simulink model "model"  (R2014a)
(part 3 of 3)

  Ответвление_от_ВЛ_110кВ_Дубовый_Лес___Островы_CN_429035693_110000_CN_296016627_110000/LConn1 -- "T_429035693__ПС_\"Островы\""/LConn1 -- Ответвление_от_ВЛ_110кВ_Дубовый_Лес___Островы_CN_429035693_110000_CN_296016647_110000/LConn1 -- Ответвление_от_ВЛ_110кВ_Дубовый_Лес___Островы_CN_429035693_110000_CN_262743896_110000/LConn1 -- Ответвление_от_ВЛ_110кВ_Дубовый_Лес___Островы_CN_429035693_110000_CN_59099213_110000/LConn1 -- Ответвление_от_ВЛ_110кВ_Дубовый_Лес___Островы_CN_429035693_110000_CN_41194024_110000/LConn1 -- Ответвление_от_ВЛ_110кВ_Дубовый_Лес___Островы_CN_429035693_110000_CN_429148816_110000/LConn1
  Ответвление_от_ВЛ_110кВ_Дубовый_Лес___Островы_CN_429035693_110000_CN_296016627_110000/LConn2 -- "T_429035693__ПС_\"Островы\""/LConn2 -- Ответвление_от_ВЛ_110кВ_Дубовый_Лес___Островы_CN_429035693_110000_CN_296016647_110000/LConn2 -- Ответвление_от_ВЛ_110кВ_Дубовый_Лес___Островы_CN_429035693_110000_CN_262743896_110000/LConn2 -- Ответвление_от_ВЛ_110кВ_Дубовый_Лес___Островы_CN_429035693_110000_CN_59099213_110000/LConn2 -- Ответвление_от_ВЛ_110кВ_Дубовый_Лес___Островы_CN_429035693_110000_CN_41194024_110000/LConn2 -- Ответвление_от_ВЛ_110кВ_Дубовый_Лес___Островы_CN_429035693_110000_CN_429148816_110000/LConn2
  Ответвление_от_ВЛ_110кВ_Дубовый_Лес___Островы_CN_429035693_110000_CN_296016627_110000/LConn3 -- "T_429035693__ПС_\"Островы\""/LConn3 -- Ответвление_от_ВЛ_110кВ_Дубовый_Лес___Островы_CN_429035693_110000_CN_296016647_110000/LConn3 -- Ответвление_от_ВЛ_110кВ_Дубовый_Лес___Островы_CN_429035693_110000_CN_262743896_110000/LConn3 -- Ответвление_от_ВЛ_110кВ_Дубовый_Лес___Островы_CN_429035693_110000_CN_59099213_110000/LConn3 -- Ответвление_от_ВЛ_110кВ_Дубовый_Лес___Островы_CN_429035693_110000_CN_41194024_110000/LConn3 -- Ответвление_от_ВЛ_110кВ_Дубовый_Лес___Островы_CN_429035693_110000_CN_429148816_110000/LConn3 -- bus12/LConn1
  "T_296016627__ПС_\"Мачулищи\""/LConn1 -- Ответвление_от_ВЛ_110кВ_Дубовый_Лес___Островы_CN_429035693_110000_CN_296016627_110000/RConn1
  "T_296016627__ПС_\"Мачулищи\""/LConn2 -- Ответвление_от_ВЛ_110кВ_Дубовый_Лес___Островы_CN_429035693_110000_CN_296016627_110000/RConn2
  Ответвление_от_ВЛ_110кВ_Дубовый_Лес___Островы_CN_429035693_110000_CN_296016627_110000/RConn3 -- "T_296016627__ПС_\"Мачулищи\""/LConn3 -- bus13/LConn1
  "T_296016647__ПС_\"Кожзавод\""/LConn1 -- Ответвление_от_ВЛ_110кВ_Дубовый_Лес___Островы_CN_429035693_110000_CN_296016647_110000/RConn1
  "T_296016647__ПС_\"Кожзавод\""/LConn2 -- Ответвление_от_ВЛ_110кВ_Дубовый_Лес___Островы_CN_429035693_110000_CN_296016647_110000/RConn2
  Ответвление_от_ВЛ_110кВ_Дубовый_Лес___Островы_CN_429035693_110000_CN_296016647_110000/RConn3 -- "T_296016647__ПС_\"Кожзавод\""/LConn3 -- bus14/LConn1
  T_262743896__/LConn1 -- Ответвление_от_ВЛ_110кВ_Дубовый_Лес___Островы_CN_429035693_110000_CN_262743896_110000/RConn1
  T_262743896__/LConn2 -- Ответвление_от_ВЛ_110кВ_Дубовый_Лес___Островы_CN_429035693_110000_CN_262743896_110000/RConn2
  Ответвление_от_ВЛ_110кВ_Дубовый_Лес___Островы_CN_429035693_110000_CN_262743896_110000/RConn3 -- T_262743896__/LConn3 -- bus15/LConn1
  "T_59099213__ПС_\"Юго_Запад\""/LConn1 -- Ответвление_от_ВЛ_110кВ_Дубовый_Лес___Островы_CN_429035693_110000_CN_59099213_110000/RConn1
  "T_59099213__ПС_\"Юго_Запад\""/LConn2 -- Ответвление_от_ВЛ_110кВ_Дубовый_Лес___Островы_CN_429035693_110000_CN_59099213_110000/RConn2
  Ответвление_от_ВЛ_110кВ_Дубовый_Лес___Островы_CN_429035693_110000_CN_59099213_110000/RConn3 -- "T_59099213__ПС_\"Юго_Запад\""/LConn3 -- bus16/LConn1
  "T_41194024__ПС_\"Курасовщина\""/LConn1 -- Ответвление_от_ВЛ_110кВ_Дубовый_Лес___Островы_CN_429035693_110000_CN_41194024_110000/RConn1
  "T_41194024__ПС_\"Курасовщина\""/LConn2 -- Ответвление_от_ВЛ_110кВ_Дубовый_Лес___Островы_CN_429035693_110000_CN_41194024_110000/RConn2
  Ответвление_от_ВЛ_110кВ_Дубовый_Лес___Островы_CN_429035693_110000_CN_41194024_110000/RConn3 -- "T_41194024__ПС_\"Курасовщина\""/LConn3 -- bus17/LConn1
  "T_429148816__ПС_\"Кока_кола\""/LConn1 -- Ответвление_от_ВЛ_110кВ_Дубовый_Лес___Островы_CN_429035693_110000_CN_429148816_110000/RConn1
  "T_429148816__ПС_\"Кока_кола\""/LConn2 -- Ответвление_от_ВЛ_110кВ_Дубовый_Лес___Островы_CN_429035693_110000_CN_429148816_110000/RConn2
  Ответвление_от_ВЛ_110кВ_Дубовый_Лес___Островы_CN_429035693_110000_CN_429148816_110000/RConn3 -- "T_429148816__ПС_\"Кока_кола\""/LConn3 -- bus18/LConn1
  T_310063635__/LConn1 -- _CN_310063635_110000_CN_310178136_110000/LConn1
  T_310063635__/LConn2 -- _CN_310063635_110000_CN_310178136_110000/LConn2
  _CN_310063635_110000_CN_310178136_110000/LConn3 -- T_310063635__/LConn3 -- bus19/LConn1
  _CN_310063635_110000_CN_310178136_110000/RConn1 -- T_310178136__/LConn1 -- _CN_245414984_110000_CN_310178136_110000/LConn1
  _CN_310063635_110000_CN_310178136_110000/RConn2 -- T_310178136__/LConn2 -- _CN_245414984_110000_CN_310178136_110000/LConn2
  _CN_310063635_110000_CN_310178136_110000/RConn3 -- T_310178136__/LConn3 -- _CN_245414984_110000_CN_310178136_110000/LConn3 -- bus20/LConn1
  T_299173918__/LConn1 -- _CN_299173918_110000_CN_240568902_110000/LConn1
  T_299173918__/LConn2 -- _CN_299173918_110000_CN_240568902_110000/LConn2
  _CN_299173918_110000_CN_240568902_110000/LConn3 -- T_299173918__/LConn3 -- bus21/LConn1
  T_240568902__/LConn1 -- _CN_299173918_110000_CN_240568902_110000/RConn1
  T_240568902__/LConn2 -- _CN_299173918_110000_CN_240568902_110000/RConn2
  _CN_299173918_110000_CN_240568902_110000/RConn3 -- T_240568902__/LConn3 -- bus22/LConn1
  _CN_287228165_110000_CN_287231999_110000/LConn1 -- T_287228165__/LConn1 -- _CN_287228165_110000_CN_130795400_110000/LConn1
  _CN_287228165_110000_CN_287231999_110000/LConn2 -- T_287228165__/LConn2 -- _CN_287228165_110000_CN_130795400_110000/LConn2
  _CN_287228165_110000_CN_287231999_110000/LConn3 -- T_287228165__/LConn3 -- _CN_287228165_110000_CN_130795400_110000/LConn3 -- bus23/LConn1
  T_287231999__/LConn1 -- _CN_287228165_110000_CN_287231999_110000/RConn1
  T_287231999__/LConn2 -- _CN_287228165_110000_CN_287231999_110000/RConn2
  _CN_287228165_110000_CN_287231999_110000/RConn3 -- T_287231999__/LConn3 -- bus24/LConn1
  T_130795400__/LConn1 -- _CN_287228165_110000_CN_130795400_110000/RConn1
  T_130795400__/LConn2 -- _CN_287228165_110000_CN_130795400_110000/RConn2
  _CN_287228165_110000_CN_130795400_110000/RConn3 -- T_130795400__/LConn3 -- bus25/LConn1
  T_237040560__/LConn1 -- _CN_237040560_110000_CN_235777846_110000/RConn1
  T_237040560__/LConn2 -- _CN_237040560_110000_CN_235777846_110000/RConn2
  _CN_237040560_110000_CN_235777846_110000/RConn3 -- T_237040560__/LConn3 -- bus26/LConn1
  T_302900770__/LConn1 -- _CN_302900770_110000_CN_314058489_110000/LConn1
  T_302900770__/LConn2 -- _CN_302900770_110000_CN_314058489_110000/LConn2
  _CN_302900770_110000_CN_314058489_110000/LConn3 -- T_302900770__/LConn3 -- bus27/LConn1
  T_314058489__/LConn1 -- _CN_302900770_110000_CN_314058489_110000/RConn1
  T_314058489__/LConn2 -- _CN_302900770_110000_CN_314058489_110000/RConn2
  _CN_302900770_110000_CN_314058489_110000/RConn3 -- T_314058489__/LConn3 -- bus28/LConn1
  _CN_288873564_110000_CN_299211088_110000/LConn1 -- T_288873564__/LConn1 -- _CN_288873564_110000_CN_288873859_110000/RConn1
  _CN_288873564_110000_CN_299211088_110000/LConn2 -- T_288873564__/LConn2 -- _CN_288873564_110000_CN_288873859_110000/RConn2
  _CN_288873564_110000_CN_299211088_110000/LConn3 -- T_288873564__/LConn3 -- _CN_288873564_110000_CN_288873859_110000/RConn3 -- bus29/LConn1
  T_299211088__/LConn1 -- _CN_288873564_110000_CN_299211088_110000/RConn1
  T_299211088__/LConn2 -- _CN_288873564_110000_CN_299211088_110000/RConn2
  _CN_288873564_110000_CN_299211088_110000/RConn3 -- T_299211088__/LConn3 -- bus30/LConn1
  "T_224125485__ПС_\"Волма\""/LConn1 -- _CN_224125485_110000_CN_429056529_110000/LConn1
  "T_224125485__ПС_\"Волма\""/LConn2 -- _CN_224125485_110000_CN_429056529_110000/LConn2
  _CN_224125485_110000_CN_429056529_110000/LConn3 -- "T_224125485__ПС_\"Волма\""/LConn3 -- bus31/LConn1
  "T_429056529__ПС_\"Сосны\""/LConn1 -- _CN_224125485_110000_CN_429056529_110000/RConn1
  "T_429056529__ПС_\"Сосны\""/LConn2 -- _CN_224125485_110000_CN_429056529_110000/RConn2
  _CN_224125485_110000_CN_429056529_110000/RConn3 -- "T_429056529__ПС_\"Сосны\""/LConn3 -- bus32/LConn1
  T_429361631__/LConn1 -- _CN_429361631_110000_CN_24423222_110000/LConn1
  T_429361631__/LConn2 -- _CN_429361631_110000_CN_24423222_110000/LConn2
  _CN_429361631_110000_CN_24423222_110000/LConn3 -- T_429361631__/LConn3 -- bus33/LConn1
  _CN_429361631_110000_CN_24423222_110000/RConn1 -- G_24423222_ТЭЦ_3/RConn1 -- _CN_417002086_110000_CN_24423222_110000/LConn1 -- _CN_399298484_110000_CN_24423222_110000/LConn1
  _CN_429361631_110000_CN_24423222_110000/RConn2 -- G_24423222_ТЭЦ_3/RConn2 -- _CN_417002086_110000_CN_24423222_110000/LConn2 -- _CN_399298484_110000_CN_24423222_110000/LConn2
  _CN_429361631_110000_CN_24423222_110000/RConn3 -- G_24423222_ТЭЦ_3/RConn3 -- _CN_417002086_110000_CN_24423222_110000/LConn3 -- _CN_399298484_110000_CN_24423222_110000/LConn3 -- bus34/LConn1
  _CN_151029302_110000_CN_229441506_110000/LConn1 -- T_151029302__ПС_17_«Сторожёвская»/LConn1 -- _CN_151029302_110000_CN_40551785_110000/LConn1 -- _CN_151029302_110000_CN_154490102_110000/LConn1 -- _CN_151029302_110000_CN_429372327_110000/LConn1 -- _CN_151029302_110000_CN_60131045_110000/LConn1
  _CN_151029302_110000_CN_229441506_110000/LConn2 -- T_151029302__ПС_17_«Сторожёвская»/LConn2 -- _CN_151029302_110000_CN_40551785_110000/LConn2 -- _CN_151029302_110000_CN_154490102_110000/LConn2 -- _CN_151029302_110000_CN_429372327_110000/LConn2 -- _CN_151029302_110000_CN_60131045_110000/LConn2
  _CN_151029302_110000_CN_229441506_110000/LConn3 -- T_151029302__ПС_17_«Сторожёвская»/LConn3 -- _CN_151029302_110000_CN_40551785_110000/LConn3 -- _CN_151029302_110000_CN_154490102_110000/LConn3 -- _CN_151029302_110000_CN_429372327_110000/LConn3 -- _CN_151029302_110000_CN_60131045_110000/LConn3 -- bus35/LConn1
  _CN_151029302_110000_CN_229441506_110000/RConn1 -- T_229441506_330000_/RConn1 -- _CN_229441505_110000_CN_229441506_110000/LConn1 -- L_229441506/LConn1
  _CN_151029302_110000_CN_229441506_110000/RConn2 -- T_229441506_330000_/RConn2 -- _CN_229441505_110000_CN_229441506_110000/LConn2 -- L_229441506/LConn2
  _CN_151029302_110000_CN_229441506_110000/RConn3 -- T_229441506_330000_/RConn3 -- _CN_229441505_110000_CN_229441506_110000/LConn3 -- L_229441506/LConn3 -- bus36/LConn1
  "T_40551785__ПС_\"Уручье\""/LConn1 -- _CN_151029302_110000_CN_40551785_110000/RConn1
  "T_40551785__ПС_\"Уручье\""/LConn2 -- _CN_151029302_110000_CN_40551785_110000/RConn2
  _CN_151029302_110000_CN_40551785_110000/RConn3 -- "T_40551785__ПС_\"Уручье\""/LConn3 -- bus37/LConn1
  G_154490102_/RConn1 -- _CN_151029302_110000_CN_154490102_110000/RConn1
  G_154490102_/RConn2 -- _CN_151029302_110000_CN_154490102_110000/RConn2
  _CN_151029302_110000_CN_154490102_110000/RConn3 -- G_154490102_/RConn3 -- bus38/LConn1
  "T_429372327__ПС_\"Дражня\""/LConn1 -- _CN_151029302_110000_CN_429372327_110000/RConn1
  "T_429372327__ПС_\"Дражня\""/LConn2 -- _CN_151029302_110000_CN_429372327_110000/RConn2
  _CN_151029302_110000_CN_429372327_110000/RConn3 -- "T_429372327__ПС_\"Дражня\""/LConn3 -- bus39/LConn1
  "T_60131045__ПС_\"Озерище\""/LConn1 -- _CN_151029302_110000_CN_60131045_110000/RConn1
  "T_60131045__ПС_\"Озерище\""/LConn2 -- _CN_151029302_110000_CN_60131045_110000/RConn2
  _CN_151029302_110000_CN_60131045_110000/RConn3 -- "T_60131045__ПС_\"Озерище\""/LConn3 -- bus40/LConn1
  _CN_300409914_110000_CN_364529034_110000/LConn1 -- T_300409914__/LConn1 -- _CN_300409914_110000_CN_247791024_110000/LConn1
  _CN_300409914_110000_CN_364529034_110000/LConn2 -- T_300409914__/LConn2 -- _CN_300409914_110000_CN_247791024_110000/LConn2
  _CN_300409914_110000_CN_364529034_110000/LConn3 -- T_300409914__/LConn3 -- _CN_300409914_110000_CN_247791024_110000/LConn3 -- bus41/LConn1
  T_364529034__/LConn1 -- _CN_300409914_110000_CN_364529034_110000/RConn1
  T_364529034__/LConn2 -- _CN_300409914_110000_CN_364529034_110000/RConn2
  _CN_300409914_110000_CN_364529034_110000/RConn3 -- T_364529034__/LConn3 -- bus42/LConn1
  _CN_300409914_110000_CN_247791024_110000/RConn1 -- "T_247791024__ПС_330кВ_\"Слуцк\""/RConn1 -- _CN_300183354_110000_CN_247791024_110000/LConn1 -- _CN_394798987_110000_CN_247791024_110000/LConn1 -- L_247791024/LConn1 -- _CN_310325079_110000_CN_247791024_110000/LConn1
  _CN_300409914_110000_CN_247791024_110000/RConn2 -- "T_247791024__ПС_330кВ_\"Слуцк\""/RConn2 -- _CN_300183354_110000_CN_247791024_110000/LConn2 -- _CN_394798987_110000_CN_247791024_110000/LConn2 -- L_247791024/LConn2 -- _CN_310325079_110000_CN_247791024_110000/LConn2
  _CN_300409914_110000_CN_247791024_110000/RConn3 -- "T_247791024__ПС_330кВ_\"Слуцк\""/RConn3 -- _CN_300183354_110000_CN_247791024_110000/LConn3 -- _CN_394798987_110000_CN_247791024_110000/LConn3 -- L_247791024/LConn3 -- bus43/LConn1 -- _CN_310325079_110000_CN_247791024_110000/LConn3
  _CN_171987005_110000_CN_173944054_110000/LConn1 -- T_171987005_330000;110000;fixme_/RConn1 -- L_171987005/LConn1
  _CN_171987005_110000_CN_173944054_110000/LConn2 -- T_171987005_330000;110000;fixme_/RConn2 -- L_171987005/LConn2
  _CN_171987005_110000_CN_173944054_110000/LConn3 -- T_171987005_330000;110000;fixme_/RConn3 -- L_171987005/LConn3 -- bus44/LConn1
  _CN_171987005_110000_CN_173944054_110000/RConn1 -- T_173944054__/LConn1 -- _CN_173944047_110000_CN_173944054_110000/LConn1
  _CN_171987005_110000_CN_173944054_110000/RConn2 -- T_173944054__/LConn2 -- _CN_173944047_110000_CN_173944054_110000/LConn2
  _CN_171987005_110000_CN_173944054_110000/RConn3 -- T_173944054__/LConn3 -- _CN_173944047_110000_CN_173944054_110000/LConn3 -- bus45/LConn1
  T_429929483__/LConn1 -- _CN_429929483_110000_CN_301229003_110000/LConn1
  T_429929483__/LConn2 -- _CN_429929483_110000_CN_301229003_110000/LConn2
  _CN_429929483_110000_CN_301229003_110000/LConn3 -- T_429929483__/LConn3 -- bus46/LConn1
  T_301229003__/LConn1 -- _CN_429929483_110000_CN_301229003_110000/RConn1
  T_301229003__/LConn2 -- _CN_429929483_110000_CN_301229003_110000/RConn2
  _CN_429929483_110000_CN_301229003_110000/RConn3 -- T_301229003__/LConn3 -- bus47/LConn1
  T_299231301__/LConn1 -- _CN_299231301_110000_CN_299226289_110000/LConn1
  T_299231301__/LConn2 -- _CN_299231301_110000_CN_299226289_110000/LConn2
  _CN_299231301_110000_CN_299226289_110000/LConn3 -- T_299231301__/LConn3 -- bus48/LConn1
  _CN_299231301_110000_CN_299226289_110000/RConn1 -- T_299226289__/LConn1 -- _CN_299226289_110000_CN_223342356_110000/LConn1
  _CN_299231301_110000_CN_299226289_110000/RConn2 -- T_299226289__/LConn2 -- _CN_299226289_110000_CN_223342356_110000/LConn2
  _CN_299231301_110000_CN_299226289_110000/RConn3 -- T_299226289__/LConn3 -- _CN_299226289_110000_CN_223342356_110000/LConn3 -- bus49/LConn1
  _CN_245414984_110000_CN_310178136_110000/RConn1 -- "T_245414984__Подстанция_330_кВ_\"Молодечно\""/RConn1 -- L_245414984/LConn1
  _CN_245414984_110000_CN_310178136_110000/RConn2 -- "T_245414984__Подстанция_330_кВ_\"Молодечно\""/RConn2 -- L_245414984/LConn2
  _CN_245414984_110000_CN_310178136_110000/RConn3 -- "T_245414984__Подстанция_330_кВ_\"Молодечно\""/RConn3 -- L_245414984/LConn3 -- bus50/LConn1
  T_263648841__/LConn1 -- _CN_263648841_110000_CN_268654506_110000/LConn1
  T_263648841__/LConn2 -- _CN_263648841_110000_CN_268654506_110000/LConn2
  _CN_263648841_110000_CN_268654506_110000/LConn3 -- T_263648841__/LConn3 -- bus51/LConn1
  T_268654506__/LConn1 -- _CN_263648841_110000_CN_268654506_110000/RConn1
  T_268654506__/LConn2 -- _CN_263648841_110000_CN_268654506_110000/RConn2
  _CN_263648841_110000_CN_268654506_110000/RConn3 -- T_268654506__/LConn3 -- bus52/LConn1
  _CN_302733791_110000_CN_302726346_110000/LConn1 -- T_302733791__/LConn1 -- _CN_302733791_110000_CN_302734379_110000/LConn1
  _CN_302733791_110000_CN_302726346_110000/LConn2 -- T_302733791__/LConn2 -- _CN_302733791_110000_CN_302734379_110000/LConn2
  _CN_302733791_110000_CN_302726346_110000/LConn3 -- T_302733791__/LConn3 -- _CN_302733791_110000_CN_302734379_110000/LConn3 -- bus53/LConn1
  T_302726346_110000_Северная/LConn1 -- _CN_302733791_110000_CN_302726346_110000/RConn1
  T_302726346_110000_Северная/LConn2 -- _CN_302733791_110000_CN_302726346_110000/RConn2
  _CN_302733791_110000_CN_302726346_110000/RConn3 -- T_302726346_110000_Северная/LConn3 -- bus54/LConn1
  T_302734379__/LConn1 -- _CN_302733791_110000_CN_302734379_110000/RConn1
  T_302734379__/LConn2 -- _CN_302733791_110000_CN_302734379_110000/RConn2
  _CN_302733791_110000_CN_302734379_110000/RConn3 -- T_302734379__/LConn3 -- bus55/LConn1
  _CN_288267865_110000_CN_295775463_110000/LConn1 -- T_288267865__/LConn1 -- _CN_288267865_110000_CN_289493943_110000/LConn1 -- _CN_288267865_110000_CN_289501225_110000/LConn1
  _CN_288267865_110000_CN_295775463_110000/LConn2 -- T_288267865__/LConn2 -- _CN_288267865_110000_CN_289493943_110000/LConn2 -- _CN_288267865_110000_CN_289501225_110000/LConn2
  _CN_288267865_110000_CN_295775463_110000/LConn3 -- T_288267865__/LConn3 -- _CN_288267865_110000_CN_289493943_110000/LConn3 -- _CN_288267865_110000_CN_289501225_110000/LConn3 -- bus56/LConn1
  T_295775463__/LConn1 -- _CN_288267865_110000_CN_295775463_110000/RConn1
  T_295775463__/LConn2 -- _CN_288267865_110000_CN_295775463_110000/RConn2
  _CN_288267865_110000_CN_295775463_110000/RConn3 -- T_295775463__/LConn3 -- bus57/LConn1
  _CN_288267865_110000_CN_289493943_110000/RConn1 -- T_289493943__РЭС/LConn1 -- _CN_289501225_110000_CN_289493943_110000/LConn1
  _CN_288267865_110000_CN_289493943_110000/RConn2 -- T_289493943__РЭС/LConn2 -- _CN_289501225_110000_CN_289493943_110000/LConn2
  _CN_288267865_110000_CN_289493943_110000/RConn3 -- T_289493943__РЭС/LConn3 -- _CN_289501225_110000_CN_289493943_110000/LConn3 -- bus58/LConn1
  _CN_288267865_110000_CN_289501225_110000/RConn1 -- T_289501225__/LConn1 -- _CN_289501225_110000_CN_289493943_110000/RConn1
  _CN_288267865_110000_CN_289501225_110000/RConn2 -- T_289501225__/LConn2 -- _CN_289501225_110000_CN_289493943_110000/RConn2
  _CN_288267865_110000_CN_289501225_110000/RConn3 -- T_289501225__/LConn3 -- _CN_289501225_110000_CN_289493943_110000/RConn3 -- bus59/LConn1
  "T_255157340__Stacja_elektroenergetyczna_110kV_\"Hołowczyce\""/LConn1 -- 110_kV_Hołowczyce___Janów_Podlaski_CN_255157340_110000_CN_110512784_110000/LConn1
  "T_255157340__Stacja_elektroenergetyczna_110kV_\"Hołowczyce\""/LConn2 -- 110_kV_Hołowczyce___Janów_Podlaski_CN_255157340_110000_CN_110512784_110000/LConn2
  110_kV_Hołowczyce___Janów_Podlaski_CN_255157340_110000_CN_110512784_110000/LConn3 -- "T_255157340__Stacja_elektroenergetyczna_110kV_\"Hołowczyce\""/LConn3 -- bus60/LConn1
  110_kV_Hołowczyce___Janów_Podlaski_CN_255157340_110000_CN_110512784_110000/RConn1 -- "T_110512784__Stacja_elektroenergetyczna_110kV_\"Janów_Podlaski\""/LConn1 -- 110_kV_Wólka_Dobryńska___Janów_Podlaski_CN_110512784_110000_CN_108158175_110000/LConn1
  110_kV_Hołowczyce___Janów_Podlaski_CN_255157340_110000_CN_110512784_110000/RConn2 -- "T_110512784__Stacja_elektroenergetyczna_110kV_\"Janów_Podlaski\""/LConn2 -- 110_kV_Wólka_Dobryńska___Janów_Podlaski_CN_110512784_110000_CN_108158175_110000/LConn2
  110_kV_Hołowczyce___Janów_Podlaski_CN_255157340_110000_CN_110512784_110000/RConn3 -- "T_110512784__Stacja_elektroenergetyczna_110kV_\"Janów_Podlaski\""/LConn3 -- 110_kV_Wólka_Dobryńska___Janów_Podlaski_CN_110512784_110000_CN_108158175_110000/LConn3 -- bus61/LConn1
  _CN_310325079_110000_CN_300419261_110000/LConn1 -- T_310325079__ПС_110_кВ_«Копыль»/LConn1 -- _CN_310325079_110000_CN_247791024_110000/RConn1 -- _CN_310325079_110000_CN_300416246_110000/LConn1
  _CN_310325079_110000_CN_300419261_110000/LConn2 -- T_310325079__ПС_110_кВ_«Копыль»/LConn2 -- _CN_310325079_110000_CN_247791024_110000/RConn2 -- _CN_310325079_110000_CN_300416246_110000/LConn2
  _CN_310325079_110000_CN_300419261_110000/LConn3 -- T_310325079__ПС_110_кВ_«Копыль»/LConn3 -- _CN_310325079_110000_CN_247791024_110000/RConn3 -- _CN_310325079_110000_CN_300416246_110000/LConn3 -- bus62/LConn1
  "T_300419261__ПС_110_кВ_\"Терасполь\""/LConn1 -- _CN_310325079_110000_CN_300419261_110000/RConn1
  "T_300419261__ПС_110_кВ_\"Терасполь\""/LConn2 -- _CN_310325079_110000_CN_300419261_110000/RConn2
  _CN_310325079_110000_CN_300419261_110000/RConn3 -- "T_300419261__ПС_110_кВ_\"Терасполь\""/LConn3 -- bus63/LConn1
  _CN_310325079_110000_CN_300416246_110000/RConn1 -- T_300416246__/LConn1 -- _CN_300416246_110000_CN_275034427_110000/LConn1
  _CN_310325079_110000_CN_300416246_110000/RConn2 -- T_300416246__/LConn2 -- _CN_300416246_110000_CN_275034427_110000/LConn2
  _CN_310325079_110000_CN_300416246_110000/RConn3 -- T_300416246__/LConn3 -- _CN_300416246_110000_CN_275034427_110000/LConn3 -- bus64/LConn1
  T_299972194__/LConn1 -- _CN_299972194_110000_CN_299960721_110000/LConn1
  T_299972194__/LConn2 -- _CN_299972194_110000_CN_299960721_110000/LConn2
  _CN_299972194_110000_CN_299960721_110000/LConn3 -- T_299972194__/LConn3 -- bus65/LConn1
  T_299960721__/LConn1 -- _CN_299972194_110000_CN_299960721_110000/RConn1
  T_299960721__/LConn2 -- _CN_299972194_110000_CN_299960721_110000/RConn2
  _CN_299972194_110000_CN_299960721_110000/RConn3 -- T_299960721__/LConn3 -- bus66/LConn1
  _CN_417002086_110000_CN_429868839_110000/LConn1 -- "T_417002086_110000_ПС_\"Корзюки\""/LConn1 -- _CN_417002086_110000_CN_24423222_110000/RConn1 -- _CN_417002086_110000_CN_429740435_110000/LConn1 -- _CN_417002086_110000_CN_429148815_110000/LConn1
  _CN_417002086_110000_CN_429868839_110000/LConn2 -- "T_417002086_110000_ПС_\"Корзюки\""/LConn2 -- _CN_417002086_110000_CN_24423222_110000/RConn2 -- _CN_417002086_110000_CN_429740435_110000/LConn2 -- _CN_417002086_110000_CN_429148815_110000/LConn2
  _CN_417002086_110000_CN_429868839_110000/LConn3 -- "T_417002086_110000_ПС_\"Корзюки\""/LConn3 -- _CN_417002086_110000_CN_24423222_110000/RConn3 -- _CN_417002086_110000_CN_429740435_110000/LConn3 -- _CN_417002086_110000_CN_429148815_110000/LConn3 -- bus67/LConn1
  T_429868839__/LConn1 -- _CN_417002086_110000_CN_429868839_110000/RConn1
  T_429868839__/LConn2 -- _CN_417002086_110000_CN_429868839_110000/RConn2
  _CN_417002086_110000_CN_429868839_110000/RConn3 -- T_429868839__/LConn3 -- bus68/LConn1
  T_429740435__/LConn1 -- _CN_417002086_110000_CN_429740435_110000/RConn1
  T_429740435__/LConn2 -- _CN_417002086_110000_CN_429740435_110000/RConn2
  _CN_417002086_110000_CN_429740435_110000/RConn3 -- T_429740435__/LConn3 -- bus69/LConn1
  T_429148815__/LConn1 -- _CN_417002086_110000_CN_429148815_110000/RConn1
  T_429148815__/LConn2 -- _CN_417002086_110000_CN_429148815_110000/RConn2
  _CN_417002086_110000_CN_429148815_110000/RConn3 -- T_429148815__/LConn3 -- bus70/LConn1
  _CN_301876843_110000_CN_296183529_110000/LConn1 -- T_301876843__/LConn1 -- _CN_301876843_110000_CN_192882077_110000/LConn1
  _CN_301876843_110000_CN_296183529_110000/LConn2 -- T_301876843__/LConn2 -- _CN_301876843_110000_CN_192882077_110000/LConn2
  _CN_301876843_110000_CN_296183529_110000/LConn3 -- T_301876843__/LConn3 -- _CN_301876843_110000_CN_192882077_110000/LConn3 -- bus71/LConn1
  T_296183529__/LConn1 -- _CN_301876843_110000_CN_296183529_110000/RConn1
  T_296183529__/LConn2 -- _CN_301876843_110000_CN_296183529_110000/RConn2
  _CN_301876843_110000_CN_296183529_110000/RConn3 -- T_296183529__/LConn3 -- bus72/LConn1
  _CN_301876843_110000_CN_192882077_110000/RConn1 -- T_192882077__/RConn1 -- L_192882077/LConn1
  _CN_301876843_110000_CN_192882077_110000/RConn2 -- T_192882077__/RConn2 -- L_192882077/LConn2
  _CN_301876843_110000_CN_192882077_110000/RConn3 -- T_192882077__/RConn3 -- L_192882077/LConn3 -- bus73/LConn1
  _CN_222038644_110000_CN_429035699_110000/LConn1 -- "T_222038644__ПС_\"Свислочь\""/LConn1 -- _CN_222038644_110000_CN_226901999_110000/LConn1 -- _CN_222038644_110000_CN_299263429_110000/LConn1
  _CN_222038644_110000_CN_429035699_110000/LConn2 -- "T_222038644__ПС_\"Свислочь\""/LConn2 -- _CN_222038644_110000_CN_226901999_110000/LConn2 -- _CN_222038644_110000_CN_299263429_110000/LConn2
  _CN_222038644_110000_CN_429035699_110000/LConn3 -- "T_222038644__ПС_\"Свислочь\""/LConn3 -- _CN_222038644_110000_CN_226901999_110000/LConn3 -- _CN_222038644_110000_CN_299263429_110000/LConn3 -- bus74/LConn1
  _CN_222038644_110000_CN_429035699_110000/RConn1 -- "T_429035699__ПС_\"СУ_ТЭЦ_5\""/LConn1 -- _CN_299263429_110000_CN_429035699_110000/LConn1
  _CN_222038644_110000_CN_429035699_110000/RConn2 -- "T_429035699__ПС_\"СУ_ТЭЦ_5\""/LConn2 -- _CN_299263429_110000_CN_429035699_110000/LConn2
  _CN_222038644_110000_CN_429035699_110000/RConn3 -- "T_429035699__ПС_\"СУ_ТЭЦ_5\""/LConn3 -- _CN_299263429_110000_CN_429035699_110000/LConn3 -- bus75/LConn1
  "T_226901999__ПС_\"Руденск\""/LConn1 -- _CN_222038644_110000_CN_226901999_110000/RConn1
  "T_226901999__ПС_\"Руденск\""/LConn2 -- _CN_222038644_110000_CN_226901999_110000/RConn2
  _CN_222038644_110000_CN_226901999_110000/RConn3 -- "T_226901999__ПС_\"Руденск\""/LConn3 -- bus76/LConn1
  _CN_222038644_110000_CN_299263429_110000/RConn1 -- T_299263429__/LConn1 -- _CN_299263429_110000_CN_429035699_110000/RConn1
  _CN_222038644_110000_CN_299263429_110000/RConn2 -- T_299263429__/LConn2 -- _CN_299263429_110000_CN_429035699_110000/RConn2
  _CN_222038644_110000_CN_299263429_110000/RConn3 -- T_299263429__/LConn3 -- _CN_299263429_110000_CN_429035699_110000/RConn3 -- bus77/LConn1
  T_296414541__/LConn1 -- _CN_296414541_110000_CN_289722224_110000/LConn1
  T_296414541__/LConn2 -- _CN_296414541_110000_CN_289722224_110000/LConn2
  _CN_296414541_110000_CN_289722224_110000/LConn3 -- T_296414541__/LConn3 -- bus78/LConn1
  _CN_296414541_110000_CN_289722224_110000/RConn1 -- T_289722224__/LConn1 -- _CN_289722224_110000_CN_25141415_110000/LConn1
  _CN_296414541_110000_CN_289722224_110000/RConn2 -- T_289722224__/LConn2 -- _CN_289722224_110000_CN_25141415_110000/LConn2
  _CN_296414541_110000_CN_289722224_110000/RConn3 -- T_289722224__/LConn3 -- _CN_289722224_110000_CN_25141415_110000/LConn3 -- bus79/LConn1
  T_294809961__/LConn1 -- _CN_294809961_110000_CN_287057886_110000/LConn1
  T_294809961__/LConn2 -- _CN_294809961_110000_CN_287057886_110000/LConn2
  _CN_294809961_110000_CN_287057886_110000/LConn3 -- T_294809961__/LConn3 -- bus80/LConn1
  T_287057886__/LConn1 -- _CN_294809961_110000_CN_287057886_110000/RConn1
  T_287057886__/LConn2 -- _CN_294809961_110000_CN_287057886_110000/RConn2
  _CN_294809961_110000_CN_287057886_110000/RConn3 -- T_287057886__/LConn3 -- bus81/LConn1
  T_34327162__/LConn1 -- _CN_34327162_110000_CN_177731028_110000/LConn1
  T_34327162__/LConn2 -- _CN_34327162_110000_CN_177731028_110000/LConn2
  _CN_34327162_110000_CN_177731028_110000/LConn3 -- T_34327162__/LConn3 -- bus82/LConn1
  _CN_34327162_110000_CN_177731028_110000/RConn1 -- T_177731028__/LConn1 -- ВЛ_110_кВ_Пилюки_Лозы_CN_89723141_110000_CN_177731028_110000/RConn1
  _CN_34327162_110000_CN_177731028_110000/RConn2 -- T_177731028__/LConn2 -- ВЛ_110_кВ_Пилюки_Лозы_CN_89723141_110000_CN_177731028_110000/RConn2
  _CN_34327162_110000_CN_177731028_110000/RConn3 -- T_177731028__/LConn3 -- ВЛ_110_кВ_Пилюки_Лозы_CN_89723141_110000_CN_177731028_110000/RConn3 -- bus83/LConn1
  T_194912891__Stacja_elektroenergetyczna_110_15_kV_Lubień/LConn1 -- Linia_110_kV_Włodawa___Lubień_CN_194912891_110000_CN_105490801_110000/LConn1
  T_194912891__Stacja_elektroenergetyczna_110_15_kV_Lubień/LConn2 -- Linia_110_kV_Włodawa___Lubień_CN_194912891_110000_CN_105490801_110000/LConn2
  Linia_110_kV_Włodawa___Lubień_CN_194912891_110000_CN_105490801_110000/LConn3 -- T_194912891__Stacja_elektroenergetyczna_110_15_kV_Lubień/LConn3 -- bus84/LConn1
  Linia_110_kV_Włodawa___Lubień_CN_194912891_110000_CN_105490801_110000/RConn1 -- T_105490801__Stacja_elektroenergetyczna_110_15_kV_Włodawa/LConn1 -- Linia_110_kV_Macoszyn___Włodawa_CN_194911376_110000_CN_105490801_110000/LConn1
  Linia_110_kV_Włodawa___Lubień_CN_194912891_110000_CN_105490801_110000/RConn2 -- T_105490801__Stacja_elektroenergetyczna_110_15_kV_Włodawa/LConn2 -- Linia_110_kV_Macoszyn___Włodawa_CN_194911376_110000_CN_105490801_110000/LConn2
  Linia_110_kV_Włodawa___Lubień_CN_194912891_110000_CN_105490801_110000/RConn3 -- T_105490801__Stacja_elektroenergetyczna_110_15_kV_Włodawa/LConn3 -- Linia_110_kV_Macoszyn___Włodawa_CN_194911376_110000_CN_105490801_110000/LConn3 -- bus85/LConn1
  T_230273156__/LConn1 -- _CN_230273156_110000_CN_230273164_110000/LConn1
  T_230273156__/LConn2 -- _CN_230273156_110000_CN_230273164_110000/LConn2
  _CN_230273156_110000_CN_230273164_110000/LConn3 -- T_230273156__/LConn3 -- bus86/LConn1
  T_230273164_110000_Подстанция_110_кВ_Южная/LConn1 -- _CN_230273156_110000_CN_230273164_110000/RConn1
  T_230273164_110000_Подстанция_110_кВ_Южная/LConn2 -- _CN_230273156_110000_CN_230273164_110000/RConn2
  _CN_230273156_110000_CN_230273164_110000/RConn3 -- T_230273164_110000_Подстанция_110_кВ_Южная/LConn3 -- bus87/LConn1
  "T_142803081__ПС_\"Заславль\""/LConn1 -- _CN_142803081_110000_CN_429035686_110000/LConn1
  "T_142803081__ПС_\"Заславль\""/LConn2 -- _CN_142803081_110000_CN_429035686_110000/LConn2
  _CN_142803081_110000_CN_429035686_110000/LConn3 -- "T_142803081__ПС_\"Заславль\""/LConn3 -- bus88/LConn1
  "T_429035686__ПС_\"Мехкарьер\""/LConn1 -- _CN_142803081_110000_CN_429035686_110000/RConn1
  "T_429035686__ПС_\"Мехкарьер\""/LConn2 -- _CN_142803081_110000_CN_429035686_110000/RConn2
  _CN_142803081_110000_CN_429035686_110000/RConn3 -- "T_429035686__ПС_\"Мехкарьер\""/LConn3 -- bus89/LConn1
  "T_108158175__Stacja_elektroenergetyczna_110kV_\"Wólka_Dobryńska\""/LConn1 -- 110_kV_Wólka_Dobryńska___Janów_Podlaski_CN_110512784_110000_CN_108158175_110000/RConn1
  "T_108158175__Stacja_elektroenergetyczna_110kV_\"Wólka_Dobryńska\""/LConn2 -- 110_kV_Wólka_Dobryńska___Janów_Podlaski_CN_110512784_110000_CN_108158175_110000/RConn2
  110_kV_Wólka_Dobryńska___Janów_Podlaski_CN_110512784_110000_CN_108158175_110000/RConn3 -- "T_108158175__Stacja_elektroenergetyczna_110kV_\"Wólka_Dobryńska\""/LConn3 -- bus90/LConn1
  "T_248455324__ПС_\"Атлант\""/LConn1 -- _CN_248455324_110000_CN_248452429_110000/LConn1
  "T_248455324__ПС_\"Атлант\""/LConn2 -- _CN_248455324_110000_CN_248452429_110000/LConn2
  _CN_248455324_110000_CN_248452429_110000/LConn3 -- "T_248455324__ПС_\"Атлант\""/LConn3 -- bus91/LConn1
  "T_248452429__ПС_\"Шабаны_2\""/LConn1 -- _CN_248455324_110000_CN_248452429_110000/RConn1
  "T_248452429__ПС_\"Шабаны_2\""/LConn2 -- _CN_248455324_110000_CN_248452429_110000/RConn2
  _CN_248455324_110000_CN_248452429_110000/RConn3 -- "T_248452429__ПС_\"Шабаны_2\""/LConn3 -- bus92/LConn1
  T_227158696__/LConn1 -- _CN_227158696_110000_CN_240810375_110000/LConn1
  T_227158696__/LConn2 -- _CN_227158696_110000_CN_240810375_110000/LConn2
  _CN_227158696_110000_CN_240810375_110000/LConn3 -- T_227158696__/LConn3 -- bus93/LConn1
  T_240810375__/LConn1 -- _CN_227158696_110000_CN_240810375_110000/RConn1
  T_240810375__/LConn2 -- _CN_227158696_110000_CN_240810375_110000/RConn2
  _CN_227158696_110000_CN_240810375_110000/RConn3 -- T_240810375__/LConn3 -- bus94/LConn1
  ВЛ_110_кВ_Лучники___Новое_Гутково_CN_373095383_110000_CN_300430643_110000/LConn1 -- T_373095383__/LConn1 -- ВЛ_110_кВ_Старые_Дороги___Новое_Гутково_CN_373095383_110000_CN_260356877_110000/LConn1
  ВЛ_110_кВ_Лучники___Новое_Гутково_CN_373095383_110000_CN_300430643_110000/LConn2 -- T_373095383__/LConn2 -- ВЛ_110_кВ_Старые_Дороги___Новое_Гутково_CN_373095383_110000_CN_260356877_110000/LConn2
  ВЛ_110_кВ_Лучники___Новое_Гутково_CN_373095383_110000_CN_300430643_110000/LConn3 -- T_373095383__/LConn3 -- ВЛ_110_кВ_Старые_Дороги___Новое_Гутково_CN_373095383_110000_CN_260356877_110000/LConn3 -- bus95/LConn1
  "T_300430643__ПС_110_кВ_\"Лучники\""/LConn1 -- ВЛ_110_кВ_Лучники___Новое_Гутково_CN_373095383_110000_CN_300430643_110000/RConn1
  "T_300430643__ПС_110_кВ_\"Лучники\""/LConn2 -- ВЛ_110_кВ_Лучники___Новое_Гутково_CN_373095383_110000_CN_300430643_110000/RConn2
  ВЛ_110_кВ_Лучники___Новое_Гутково_CN_373095383_110000_CN_300430643_110000/RConn3 -- "T_300430643__ПС_110_кВ_\"Лучники\""/LConn3 -- bus96/LConn1
  ВЛ_110_кВ_Старые_Дороги___Новое_Гутково_CN_373095383_110000_CN_260356877_110000/RConn1 -- T_260356877_750000;330000_Белорусская/RConn1 -- L_260356877/LConn1
  ВЛ_110_кВ_Старые_Дороги___Новое_Гутково_CN_373095383_110000_CN_260356877_110000/RConn2 -- T_260356877_750000;330000_Белорусская/RConn2 -- L_260356877/LConn2
  ВЛ_110_кВ_Старые_Дороги___Новое_Гутково_CN_373095383_110000_CN_260356877_110000/RConn3 -- T_260356877_750000;330000_Белорусская/RConn3 -- L_260356877/LConn3 -- bus97/LConn1
  T_223342356__/LConn1 -- _CN_299226289_110000_CN_223342356_110000/RConn1
  T_223342356__/LConn2 -- _CN_299226289_110000_CN_223342356_110000/RConn2
  _CN_299226289_110000_CN_223342356_110000/RConn3 -- T_223342356__/LConn3 -- bus98/LConn1
  T_409058996__/LConn1 -- ВЛ_Калийная___Уречье_110кВ_CN_409058996_110000_CN_232431375_110000/LConn1
  T_409058996__/LConn2 -- ВЛ_Калийная___Уречье_110кВ_CN_409058996_110000_CN_232431375_110000/LConn2
  ВЛ_Калийная___Уречье_110кВ_CN_409058996_110000_CN_232431375_110000/LConn3 -- T_409058996__/LConn3 -- bus99/LConn1
  T_232431375__/LConn1 -- ВЛ_Калийная___Уречье_110кВ_CN_409058996_110000_CN_232431375_110000/RConn1
  T_232431375__/LConn2 -- ВЛ_Калийная___Уречье_110кВ_CN_409058996_110000_CN_232431375_110000/RConn2
  ВЛ_Калийная___Уречье_110кВ_CN_409058996_110000_CN_232431375_110000/RConn3 -- T_232431375__/LConn3 -- bus100/LConn1
  _CN_283245238_110000_CN_235391296_110000/LConn1 -- T_283245238_330000_/RConn1 -- L_283245238/LConn1
  _CN_283245238_110000_CN_235391296_110000/LConn2 -- T_283245238_330000_/RConn2 -- L_283245238/LConn2
  _CN_283245238_110000_CN_235391296_110000/LConn3 -- T_283245238_330000_/RConn3 -- L_283245238/LConn3 -- bus101/LConn1
  _CN_283245238_110000_CN_235391296_110000/RConn1 -- T_235391296__/LConn1 -- _CN_235777846_110000_CN_235391296_110000/RConn1
  _CN_283245238_110000_CN_235391296_110000/RConn2 -- T_235391296__/LConn2 -- _CN_235777846_110000_CN_235391296_110000/RConn2
  _CN_283245238_110000_CN_235391296_110000/RConn3 -- T_235391296__/LConn3 -- _CN_235777846_110000_CN_235391296_110000/RConn3 -- bus102/LConn1
  "T_275034427__ПС_\"Красная_Слобода\""/LConn1 -- _CN_300416246_110000_CN_275034427_110000/RConn1
  "T_275034427__ПС_\"Красная_Слобода\""/LConn2 -- _CN_300416246_110000_CN_275034427_110000/RConn2
  _CN_300416246_110000_CN_275034427_110000/RConn3 -- "T_275034427__ПС_\"Красная_Слобода\""/LConn3 -- bus103/LConn1
  T_309889740__/LConn1 -- _CN_309889740_110000_CN_25141415_110000/LConn1
  T_309889740__/LConn2 -- _CN_309889740_110000_CN_25141415_110000/LConn2
  _CN_309889740_110000_CN_25141415_110000/LConn3 -- T_309889740__/LConn3 -- bus104/LConn1
  _CN_309889740_110000_CN_25141415_110000/RConn1 -- G_25141415_Берёзовская_ГРЭС/RConn1 -- _CN_289722224_110000_CN_25141415_110000/RConn1 -- 220kV_Białystok___Рось_CN_216254873_220000_CN_25141415_110000/LConn1
  _CN_309889740_110000_CN_25141415_110000/RConn2 -- G_25141415_Берёзовская_ГРЭС/RConn2 -- _CN_289722224_110000_CN_25141415_110000/RConn2 -- 220kV_Białystok___Рось_CN_216254873_220000_CN_25141415_110000/LConn2
  _CN_309889740_110000_CN_25141415_110000/RConn3 -- G_25141415_Берёзовская_ГРЭС/RConn3 -- _CN_289722224_110000_CN_25141415_110000/RConn3 -- 220kV_Białystok___Рось_CN_216254873_220000_CN_25141415_110000/LConn3 -- bus105/LConn1
  _CN_230054607_110000_CN_271931809_110000/LConn1 -- T_230054607__Барановичи_330/RConn4 -- _CN_230054607_110000_CN_296408783_110000/LConn1 -- _CN_230054607_110000_CN_230054608_110000/LConn1 -- L_230054607/LConn1
  _CN_230054607_110000_CN_271931809_110000/LConn2 -- T_230054607__Барановичи_330/RConn5 -- _CN_230054607_110000_CN_296408783_110000/LConn2 -- _CN_230054607_110000_CN_230054608_110000/LConn2 -- L_230054607/LConn2
  _CN_230054607_110000_CN_271931809_110000/LConn3 -- T_230054607__Барановичи_330/RConn6 -- _CN_230054607_110000_CN_296408783_110000/LConn3 -- _CN_230054607_110000_CN_230054608_110000/LConn3 -- L_230054607/LConn3 -- bus106/LConn1
  T_271931809__/LConn1 -- _CN_230054607_110000_CN_271931809_110000/RConn1
  T_271931809__/LConn2 -- _CN_230054607_110000_CN_271931809_110000/RConn2
  _CN_230054607_110000_CN_271931809_110000/RConn3 -- T_271931809__/LConn3 -- bus107/LConn1
  T_296408783__/LConn1 -- _CN_230054607_110000_CN_296408783_110000/RConn1
  T_296408783__/LConn2 -- _CN_230054607_110000_CN_296408783_110000/RConn2
  _CN_230054607_110000_CN_296408783_110000/RConn3 -- T_296408783__/LConn3 -- bus108/LConn1
  _CN_230054607_110000_CN_230054608_110000/RConn1 -- T_230054608__Барановичи_220/RConn1 -- _CN_230054608_110000_CN_230054609_110000/LConn1 -- L_230054608/LConn1
  _CN_230054607_110000_CN_230054608_110000/RConn2 -- T_230054608__Барановичи_220/RConn2 -- _CN_230054608_110000_CN_230054609_110000/LConn2 -- L_230054608/LConn2
  _CN_230054607_110000_CN_230054608_110000/RConn3 -- T_230054608__Барановичи_220/RConn3 -- _CN_230054608_110000_CN_230054609_110000/LConn3 -- L_230054608/LConn3 -- bus109/LConn1
  T_230054609__/LConn1 -- _CN_230054608_110000_CN_230054609_110000/RConn1
  T_230054609__/LConn2 -- _CN_230054608_110000_CN_230054609_110000/RConn2
  _CN_230054608_110000_CN_230054609_110000/RConn3 -- T_230054609__/LConn3 -- bus110/LConn1
  T_298978939__/LConn1 -- _CN_298978939_110000_CN_280269221_110000/LConn1
  T_298978939__/LConn2 -- _CN_298978939_110000_CN_280269221_110000/LConn2
  _CN_298978939_110000_CN_280269221_110000/LConn3 -- T_298978939__/LConn3 -- bus111/LConn1
  T_280269221__/LConn1 -- _CN_298978939_110000_CN_280269221_110000/RConn1
  T_280269221__/LConn2 -- _CN_298978939_110000_CN_280269221_110000/RConn2
  _CN_298978939_110000_CN_280269221_110000/RConn3 -- T_280269221__/LConn3 -- bus112/LConn1
  _CN_173944047_110000_CN_311242021_110000/LConn1 -- T_173944047__/LConn1 -- _CN_173944047_110000_CN_173944054_110000/RConn1
  _CN_173944047_110000_CN_311242021_110000/LConn2 -- T_173944047__/LConn2 -- _CN_173944047_110000_CN_173944054_110000/RConn2
  _CN_173944047_110000_CN_311242021_110000/LConn3 -- T_173944047__/LConn3 -- _CN_173944047_110000_CN_173944054_110000/RConn3 -- bus113/LConn1
  T_311242021__/LConn1 -- _CN_173944047_110000_CN_311242021_110000/RConn1
  T_311242021__/LConn2 -- _CN_173944047_110000_CN_311242021_110000/RConn2
  _CN_173944047_110000_CN_311242021_110000/RConn3 -- T_311242021__/LConn3 -- bus114/LConn1
  T_192951026__/LConn1 -- _CN_192951026_110000_CN_201828730_110000/LConn1
  T_192951026__/LConn2 -- _CN_192951026_110000_CN_201828730_110000/LConn2
  _CN_192951026_110000_CN_201828730_110000/LConn3 -- T_192951026__/LConn3 -- bus115/LConn1
  _CN_192951026_110000_CN_201828730_110000/RConn1 -- T_201828730_330000_/RConn4 -- _CN_325933845_110000_CN_201828730_110000/LConn1 -- L_201828730/LConn1
  _CN_192951026_110000_CN_201828730_110000/RConn2 -- T_201828730_330000_/RConn5 -- _CN_325933845_110000_CN_201828730_110000/LConn2 -- L_201828730/LConn2
  _CN_192951026_110000_CN_201828730_110000/RConn3 -- T_201828730_330000_/RConn6 -- _CN_325933845_110000_CN_201828730_110000/LConn3 -- L_201828730/LConn3 -- bus116/LConn1
  T_168120565__/LConn1 -- _CN_168120565_110000_CN_199487387_110000/LConn1
  T_168120565__/LConn2 -- _CN_168120565_110000_CN_199487387_110000/LConn2
  _CN_168120565_110000_CN_199487387_110000/LConn3 -- T_168120565__/LConn3 -- bus117/LConn1
  T_199487387__/LConn1 -- _CN_168120565_110000_CN_199487387_110000/RConn1
  T_199487387__/LConn2 -- _CN_168120565_110000_CN_199487387_110000/RConn2
  _CN_168120565_110000_CN_199487387_110000/RConn3 -- T_199487387__/LConn3 -- bus118/LConn1
  T_223761142__ПС_110_кВ_Гродненская_ГЭС/LConn1 -- _CN_223761142_110000_CN_177731027_110000/LConn1
  T_223761142__ПС_110_кВ_Гродненская_ГЭС/LConn2 -- _CN_223761142_110000_CN_177731027_110000/LConn2
  _CN_223761142_110000_CN_177731027_110000/LConn3 -- T_223761142__ПС_110_кВ_Гродненская_ГЭС/LConn3 -- bus119/LConn1
  T_177731027__/LConn1 -- _CN_223761142_110000_CN_177731027_110000/RConn1
  T_177731027__/LConn2 -- _CN_223761142_110000_CN_177731027_110000/RConn2
  _CN_223761142_110000_CN_177731027_110000/RConn3 -- T_177731027__/LConn3 -- bus120/LConn1
  "T_52763915__ПС_\"Лошица\""/LConn1 -- _CN_52763915_110000_CN_143993676_110000/LConn1
  "T_52763915__ПС_\"Лошица\""/LConn2 -- _CN_52763915_110000_CN_143993676_110000/LConn2
  _CN_52763915_110000_CN_143993676_110000/LConn3 -- "T_52763915__ПС_\"Лошица\""/LConn3 -- bus121/LConn1
  T_143993676__ПС_Минский_камвольный_комбинат/LConn1 -- _CN_52763915_110000_CN_143993676_110000/RConn1
  T_143993676__ПС_Минский_камвольный_комбинат/LConn2 -- _CN_52763915_110000_CN_143993676_110000/RConn2
  _CN_52763915_110000_CN_143993676_110000/RConn3 -- T_143993676__ПС_Минский_камвольный_комбинат/LConn3 -- bus122/LConn1
  _CN_325933845_110000_CN_201828730_110000/RConn1 -- T_325933845__/LConn1 -- _CN_325933845_110000_CN_166169945_110000/LConn1
  _CN_325933845_110000_CN_201828730_110000/RConn2 -- T_325933845__/LConn2 -- _CN_325933845_110000_CN_166169945_110000/LConn2
  _CN_325933845_110000_CN_201828730_110000/RConn3 -- T_325933845__/LConn3 -- _CN_325933845_110000_CN_166169945_110000/LConn3 -- bus123/LConn1
  _CN_325933845_110000_CN_166169945_110000/RConn1 -- T_166169945__/LConn1 -- _CN_166169945_110000_CN_88831410_110000/LConn1
  _CN_325933845_110000_CN_166169945_110000/RConn2 -- T_166169945__/LConn2 -- _CN_166169945_110000_CN_88831410_110000/LConn2
  _CN_325933845_110000_CN_166169945_110000/RConn3 -- T_166169945__/LConn3 -- _CN_166169945_110000_CN_88831410_110000/LConn3 -- bus124/LConn1
  _CN_230059286_110000_CN_230059305_110000/LConn1 -- T_230059286__/RConn1 -- L_230059286/LConn1
  _CN_230059286_110000_CN_230059305_110000/LConn2 -- T_230059286__/RConn2 -- L_230059286/LConn2
  _CN_230059286_110000_CN_230059305_110000/LConn3 -- T_230059286__/RConn3 -- L_230059286/LConn3 -- bus125/LConn1
  _CN_230059286_110000_CN_230059305_110000/RConn1 -- T_230059305_110000_Осташковичи/LConn1 -- _CN_230059305_110000_CN_282201051_110000/LConn1
  _CN_230059286_110000_CN_230059305_110000/RConn2 -- T_230059305_110000_Осташковичи/LConn2 -- _CN_230059305_110000_CN_282201051_110000/LConn2
  _CN_230059286_110000_CN_230059305_110000/RConn3 -- T_230059305_110000_Осташковичи/LConn3 -- _CN_230059305_110000_CN_282201051_110000/LConn3 -- bus126/LConn1
  T_366740253__/LConn1 -- _CN_366740253_110000_CN_262762815_110000/LConn1
  T_366740253__/LConn2 -- _CN_366740253_110000_CN_262762815_110000/LConn2
  _CN_366740253_110000_CN_262762815_110000/LConn3 -- T_366740253__/LConn3 -- bus127/LConn1
  T_262762815__/LConn1 -- _CN_366740253_110000_CN_262762815_110000/RConn1
  T_262762815__/LConn2 -- _CN_366740253_110000_CN_262762815_110000/RConn2
  _CN_366740253_110000_CN_262762815_110000/RConn3 -- T_262762815__/LConn3 -- bus128/LConn1
  T_282201051__Якимова_Слобода/LConn1 -- _CN_230059305_110000_CN_282201051_110000/RConn1
  T_282201051__Якимова_Слобода/LConn2 -- _CN_230059305_110000_CN_282201051_110000/RConn2
  _CN_230059305_110000_CN_282201051_110000/RConn3 -- T_282201051__Якимова_Слобода/LConn3 -- bus129/LConn1
  T_282200754_110000_Забродье/LConn1 -- _CN_282200754_110000_CN_286434280_110000/LConn1
  T_282200754_110000_Забродье/LConn2 -- _CN_282200754_110000_CN_286434280_110000/LConn2
  _CN_282200754_110000_CN_286434280_110000/LConn3 -- T_282200754_110000_Забродье/LConn3 -- bus130/LConn1
  T_286434280__/LConn1 -- _CN_282200754_110000_CN_286434280_110000/RConn1
  T_286434280__/LConn2 -- _CN_282200754_110000_CN_286434280_110000/RConn2
  _CN_282200754_110000_CN_286434280_110000/RConn3 -- T_286434280__/LConn3 -- bus131/LConn1
  _CN_300183354_110000_CN_247791024_110000/RConn1 -- T_300183354__/LConn1 -- _CN_300183354_110000_CN_300236667_110000/LConn1
  _CN_300183354_110000_CN_247791024_110000/RConn2 -- T_300183354__/LConn2 -- _CN_300183354_110000_CN_300236667_110000/LConn2
  _CN_300183354_110000_CN_247791024_110000/RConn3 -- T_300183354__/LConn3 -- _CN_300183354_110000_CN_300236667_110000/LConn3 -- bus132/LConn1
  T_300236667__/LConn1 -- _CN_300183354_110000_CN_300236667_110000/RConn1
  T_300236667__/LConn2 -- _CN_300183354_110000_CN_300236667_110000/RConn2
  _CN_300183354_110000_CN_300236667_110000/RConn3 -- T_300236667__/LConn3 -- bus133/LConn1
  T_108689220__/LConn1 -- _CN_108689220_110000_CN_295351112_110000/LConn1
  T_108689220__/LConn2 -- _CN_108689220_110000_CN_295351112_110000/LConn2
  _CN_108689220_110000_CN_295351112_110000/LConn3 -- T_108689220__/LConn3 -- bus134/LConn1
  _CN_108689220_110000_CN_295351112_110000/RConn1 -- T_295351112_330000_/LConn1 -- _CN_295351112_110000_CN_168037760_110000/LConn1
  _CN_108689220_110000_CN_295351112_110000/RConn2 -- T_295351112_330000_/LConn2 -- _CN_295351112_110000_CN_168037760_110000/LConn2
  _CN_108689220_110000_CN_295351112_110000/RConn3 -- T_295351112_330000_/LConn3 -- _CN_295351112_110000_CN_168037760_110000/LConn3 -- bus135/LConn1
  T_168037760__/LConn1 -- _CN_295351112_110000_CN_168037760_110000/RConn1
  T_168037760__/LConn2 -- _CN_295351112_110000_CN_168037760_110000/RConn2
  _CN_295351112_110000_CN_168037760_110000/RConn3 -- T_168037760__/LConn3 -- bus136/LConn1
  _CN_293851177_110000_CN_276283812_110000/LConn1 -- T_293851177__/LConn1 -- _CN_293851177_110000_CN_293845492_110000/LConn1
  _CN_293851177_110000_CN_276283812_110000/LConn2 -- T_293851177__/LConn2 -- _CN_293851177_110000_CN_293845492_110000/LConn2
  _CN_293851177_110000_CN_276283812_110000/LConn3 -- T_293851177__/LConn3 -- _CN_293851177_110000_CN_293845492_110000/LConn3 -- bus137/LConn1
  T_276283812__/LConn1 -- _CN_293851177_110000_CN_276283812_110000/RConn1
  T_276283812__/LConn2 -- _CN_293851177_110000_CN_276283812_110000/RConn2
  _CN_293851177_110000_CN_276283812_110000/RConn3 -- T_276283812__/LConn3 -- bus138/LConn1
  T_293845492__/LConn1 -- _CN_293851177_110000_CN_293845492_110000/RConn1
  T_293845492__/LConn2 -- _CN_293851177_110000_CN_293845492_110000/RConn2
  _CN_293851177_110000_CN_293845492_110000/RConn3 -- T_293845492__/LConn3 -- bus139/LConn1
  T_88831410__/LConn1 -- _CN_166169945_110000_CN_88831410_110000/RConn1
  T_88831410__/LConn2 -- _CN_166169945_110000_CN_88831410_110000/RConn2
  _CN_166169945_110000_CN_88831410_110000/RConn3 -- T_88831410__/LConn3 -- bus140/LConn1
  T_194911376__Stacja_elektroenergetyczna_110_15_kV_Macoszyn/LConn1 -- Linia_110_kV_Macoszyn___Włodawa_CN_194911376_110000_CN_105490801_110000/RConn1
  T_194911376__Stacja_elektroenergetyczna_110_15_kV_Macoszyn/LConn2 -- Linia_110_kV_Macoszyn___Włodawa_CN_194911376_110000_CN_105490801_110000/RConn2
  Linia_110_kV_Macoszyn___Włodawa_CN_194911376_110000_CN_105490801_110000/RConn3 -- T_194911376__Stacja_elektroenergetyczna_110_15_kV_Macoszyn/LConn3 -- bus141/LConn1
  "T_25686883__ПС_\"Сухарево\""/LConn1 -- _CN_25686883_110000_CN_264555597_110000/LConn1
  "T_25686883__ПС_\"Сухарево\""/LConn2 -- _CN_25686883_110000_CN_264555597_110000/LConn2
  _CN_25686883_110000_CN_264555597_110000/LConn3 -- "T_25686883__ПС_\"Сухарево\""/LConn3 -- bus142/LConn1
  "T_264555597__ПС_\"Ждановичи\""/LConn1 -- _CN_25686883_110000_CN_264555597_110000/RConn1
  "T_264555597__ПС_\"Ждановичи\""/LConn2 -- _CN_25686883_110000_CN_264555597_110000/RConn2
  _CN_25686883_110000_CN_264555597_110000/RConn3 -- "T_264555597__ПС_\"Ждановичи\""/LConn3 -- bus143/LConn1
  T_394798987__/LConn1 -- _CN_394798987_110000_CN_247791024_110000/RConn1
  T_394798987__/LConn2 -- _CN_394798987_110000_CN_247791024_110000/RConn2
  _CN_394798987_110000_CN_247791024_110000/RConn3 -- T_394798987__/LConn3 -- bus144/LConn1
  "T_399298484_110000_ПС_\"Завод_запасных_частей\""/LConn1 -- _CN_399298484_110000_CN_24423222_110000/RConn1
  "T_399298484_110000_ПС_\"Завод_запасных_частей\""/LConn2 -- _CN_399298484_110000_CN_24423222_110000/RConn2
  _CN_399298484_110000_CN_24423222_110000/RConn3 -- "T_399298484_110000_ПС_\"Завод_запасных_частей\""/LConn3 -- bus145/LConn1
  T_39890905__/LConn1 -- _CN_39890905_110000_CN_29128697_110000/LConn1
  T_39890905__/LConn2 -- _CN_39890905_110000_CN_29128697_110000/LConn2
  _CN_39890905_110000_CN_29128697_110000/LConn3 -- T_39890905__/LConn3 -- bus146/LConn1
  T_29128697__ПС_110_кВ_Занеманская/LConn1 -- _CN_39890905_110000_CN_29128697_110000/RConn1
  T_29128697__ПС_110_кВ_Занеманская/LConn2 -- _CN_39890905_110000_CN_29128697_110000/RConn2
  _CN_39890905_110000_CN_29128697_110000/RConn3 -- T_29128697__ПС_110_кВ_Занеманская/LConn3 -- bus147/LConn1
  "T_229441505__ПС_\"Вишневка\""/LConn1 -- _CN_229441505_110000_CN_229441506_110000/RConn1
  "T_229441505__ПС_\"Вишневка\""/LConn2 -- _CN_229441505_110000_CN_229441506_110000/RConn2
  _CN_229441505_110000_CN_229441506_110000/RConn3 -- "T_229441505__ПС_\"Вишневка\""/LConn3 -- bus148/LConn1
  _CN_300347040_220000_CN_230059284_220000/LConn1 -- T_300347040_330000_/LConn1 -- _CN_300347040_220000_CN_264617753_220000/LConn1 -- _CN_300347040_220000_CN_230059286_220000/LConn1
  _CN_300347040_220000_CN_230059284_220000/LConn2 -- T_300347040_330000_/LConn2 -- _CN_300347040_220000_CN_264617753_220000/LConn2 -- _CN_300347040_220000_CN_230059286_220000/LConn2
  _CN_300347040_220000_CN_230059284_220000/LConn3 -- T_300347040_330000_/LConn3 -- _CN_300347040_220000_CN_264617753_220000/LConn3 -- _CN_300347040_220000_CN_230059286_220000/LConn3 -- bus149/LConn1
  T_230059284__/LConn1 -- _CN_300347040_220000_CN_230059284_220000/RConn1
  T_230059284__/LConn2 -- _CN_300347040_220000_CN_230059284_220000/RConn2
  _CN_300347040_220000_CN_230059284_220000/RConn3 -- T_230059284__/LConn3 -- bus150/LConn1
  _CN_300347040_220000_CN_264617753_220000/RConn1 -- T_264617753__РЭС/LConn1 -- _CN_287216880_220000_CN_264617753_220000/LConn1
  _CN_300347040_220000_CN_264617753_220000/RConn2 -- T_264617753__РЭС/LConn2 -- _CN_287216880_220000_CN_264617753_220000/LConn2
  _CN_300347040_220000_CN_264617753_220000/RConn3 -- T_264617753__РЭС/LConn3 -- _CN_287216880_220000_CN_264617753_220000/LConn3 -- bus151/LConn1
  T_230059286__/LConn1 -- _CN_300347040_220000_CN_230059286_220000/RConn1
  T_230059286__/LConn2 -- _CN_300347040_220000_CN_230059286_220000/RConn2
  _CN_300347040_220000_CN_230059286_220000/RConn3 -- T_230059286__/LConn3 -- bus152/LConn1
  _CN_287216880_220000_CN_264617753_220000/RConn1 -- T_287216880_330000_Гомель_330/RConn1 -- L_287216880/LConn1
  _CN_287216880_220000_CN_264617753_220000/RConn2 -- T_287216880_330000_Гомель_330/RConn2 -- L_287216880/LConn2
  _CN_287216880_220000_CN_264617753_220000/RConn3 -- T_287216880_330000_Гомель_330/RConn3 -- L_287216880/LConn3 -- bus153/LConn1
  _CN_230054607_220000_CN_230054608_220000/LConn1 -- T_230054607__Барановичи_330/RConn1 -- _CN_230054607_220000_CN_303000490_220000/LConn1
  _CN_230054607_220000_CN_230054608_220000/LConn2 -- T_230054607__Барановичи_330/RConn2 -- _CN_230054607_220000_CN_303000490_220000/LConn2
  _CN_230054607_220000_CN_230054608_220000/LConn3 -- T_230054607__Барановичи_330/RConn3 -- _CN_230054607_220000_CN_303000490_220000/LConn3 -- bus154/LConn1
  T_230054608__Барановичи_220/LConn1 -- _CN_230054607_220000_CN_230054608_220000/RConn1
  T_230054608__Барановичи_220/LConn2 -- _CN_230054607_220000_CN_230054608_220000/RConn2
  _CN_230054607_220000_CN_230054608_220000/RConn3 -- T_230054608__Барановичи_220/LConn3 -- bus155/LConn1
  _CN_230054607_220000_CN_303000490_220000/RConn1 -- T_303000490_330000_/RConn1 -- L_303000490/LConn1
  _CN_230054607_220000_CN_303000490_220000/RConn2 -- T_303000490_330000_/RConn2 -- L_303000490/LConn2
  _CN_230054607_220000_CN_303000490_220000/RConn3 -- T_303000490_330000_/RConn3 -- L_303000490/LConn3 -- bus156/LConn1
  220kV_Białystok___Рось_CN_216254873_220000_CN_201828730_220000/LConn1 -- "T_216254873_220000;110000_Stacja_elektroenergetyczna_\"Białystok\"_220_110_kV"/LConn1 -- 220kV_Białystok___Рось_CN_216254873_220000_CN_25141415_110000/RConn1
  220kV_Białystok___Рось_CN_216254873_220000_CN_201828730_220000/LConn2 -- "T_216254873_220000;110000_Stacja_elektroenergetyczna_\"Białystok\"_220_110_kV"/LConn2 -- 220kV_Białystok___Рось_CN_216254873_220000_CN_25141415_110000/RConn2
  220kV_Białystok___Рось_CN_216254873_220000_CN_201828730_220000/LConn3 -- "T_216254873_220000;110000_Stacja_elektroenergetyczna_\"Białystok\"_220_110_kV"/LConn3 -- 220kV_Białystok___Рось_CN_216254873_220000_CN_25141415_110000/RConn3 -- bus157/LConn1
  T_201828730_330000_/RConn1 -- 220kV_Białystok___Рось_CN_216254873_220000_CN_201828730_220000/RConn1
  T_201828730_330000_/RConn2 -- 220kV_Białystok___Рось_CN_216254873_220000_CN_201828730_220000/RConn2
  220kV_Białystok___Рось_CN_216254873_220000_CN_201828730_220000/RConn3 -- T_201828730_330000_/RConn3 -- bus158/LConn1
  T_129510527__/LConn1 -- _CN_129510527_220000_CN_148660895_220000/LConn1
  T_129510527__/LConn2 -- _CN_129510527_220000_CN_148660895_220000/LConn2
  _CN_129510527_220000_CN_148660895_220000/LConn3 -- T_129510527__/LConn3 -- bus159/LConn1
  T_148660895__P_C_220_kV_BREST_2/LConn1 -- _CN_129510527_220000_CN_148660895_220000/RConn1
  T_148660895__P_C_220_kV_BREST_2/LConn2 -- _CN_129510527_220000_CN_148660895_220000/RConn2
  _CN_129510527_220000_CN_148660895_220000/RConn3 -- T_148660895__P_C_220_kV_BREST_2/LConn3 -- bus160/LConn1
  T_296423596__/LConn1 -- _CN_296423596_330000_CN_303000490_330000/LConn1
  T_296423596__/LConn2 -- _CN_296423596_330000_CN_303000490_330000/LConn2
  _CN_296423596_330000_CN_303000490_330000/LConn3 -- T_296423596__/LConn3 -- bus161/LConn1
  T_303000490_330000_/LConn1 -- _CN_296423596_330000_CN_303000490_330000/RConn1
  T_303000490_330000_/LConn2 -- _CN_296423596_330000_CN_303000490_330000/RConn2
  _CN_296423596_330000_CN_303000490_330000/RConn3 -- T_303000490_330000_/LConn3 -- bus162/LConn1
  _CN_299839754_330000_CN_232797676_330000/LConn1 -- T_299839754__/LConn1 -- _CN_299839754_330000_CN_260356877_330000/LConn1
  _CN_299839754_330000_CN_232797676_330000/LConn2 -- T_299839754__/LConn2 -- _CN_299839754_330000_CN_260356877_330000/LConn2
  _CN_299839754_330000_CN_232797676_330000/LConn3 -- T_299839754__/LConn3 -- _CN_299839754_330000_CN_260356877_330000/LConn3 -- bus163/LConn1
  "T_232797676__ПС_330_\"Калийная\""/LConn1 -- _CN_299839754_330000_CN_232797676_330000/RConn1
  "T_232797676__ПС_330_\"Калийная\""/LConn2 -- _CN_299839754_330000_CN_232797676_330000/RConn2
  _CN_299839754_330000_CN_232797676_330000/RConn3 -- "T_232797676__ПС_330_\"Калийная\""/LConn3 -- bus164/LConn1
  _CN_299839754_330000_CN_260356877_330000/RConn1 -- T_260356877_750000;330000_Белорусская/LConn1 -- ВЛ_330_кВ_Белорусская___Слуцк_CN_260356877_330000_CN_247791024_330000/LConn1
  _CN_299839754_330000_CN_260356877_330000/RConn2 -- T_260356877_750000;330000_Белорусская/LConn2 -- ВЛ_330_кВ_Белорусская___Слуцк_CN_260356877_330000_CN_247791024_330000/LConn2
  _CN_299839754_330000_CN_260356877_330000/RConn3 -- T_260356877_750000;330000_Белорусская/LConn3 -- ВЛ_330_кВ_Белорусская___Слуцк_CN_260356877_330000_CN_247791024_330000/LConn3 -- bus165/LConn1
  ВЛ_330_кВ_Белорусская___Слуцк_CN_260356877_330000_CN_247791024_330000/RConn1 -- "T_247791024__ПС_330кВ_\"Слуцк\""/LConn1 -- ВЛ_330_кВ_ТЭЦ_4___Слуцк_CN_247791024_330000_CN_25465034_330000/LConn1
  ВЛ_330_кВ_Белорусская___Слуцк_CN_260356877_330000_CN_247791024_330000/RConn2 -- "T_247791024__ПС_330кВ_\"Слуцк\""/LConn2 -- ВЛ_330_кВ_ТЭЦ_4___Слуцк_CN_247791024_330000_CN_25465034_330000/LConn2
  ВЛ_330_кВ_Белорусская___Слуцк_CN_260356877_330000_CN_247791024_330000/RConn3 -- "T_247791024__ПС_330кВ_\"Слуцк\""/LConn3 -- ВЛ_330_кВ_ТЭЦ_4___Слуцк_CN_247791024_330000_CN_25465034_330000/LConn3 -- bus166/LConn1
  "T_429151634__ПС_\"Борисов\""/LConn1 -- _CN_429151634_330000_CN_405472760_330000/LConn1
  "T_429151634__ПС_\"Борисов\""/LConn2 -- _CN_429151634_330000_CN_405472760_330000/LConn2
  _CN_429151634_330000_CN_405472760_330000/LConn3 -- "T_429151634__ПС_\"Борисов\""/LConn3 -- bus167/LConn1
  _CN_429151634_330000_CN_405472760_330000/RConn1 -- "T_405472760__ПС_330_110_10_кВ_\"Восточная\""/LConn1 -- ВЛ_426_Восточная___Северная_CN_229441506_330000_CN_405472760_330000/LConn1
  _CN_429151634_330000_CN_405472760_330000/RConn2 -- "T_405472760__ПС_330_110_10_кВ_\"Восточная\""/LConn2 -- ВЛ_426_Восточная___Северная_CN_229441506_330000_CN_405472760_330000/LConn2
  _CN_429151634_330000_CN_405472760_330000/RConn3 -- "T_405472760__ПС_330_110_10_кВ_\"Восточная\""/LConn3 -- ВЛ_426_Восточная___Северная_CN_229441506_330000_CN_405472760_330000/LConn3 -- bus168/LConn1
  T_192882077__/LConn1 -- _CN_192882077_330000_CN_112459307_330000/LConn1
  T_192882077__/LConn2 -- _CN_192882077_330000_CN_112459307_330000/LConn2
  _CN_192882077_330000_CN_112459307_330000/LConn3 -- T_192882077__/LConn3 -- bus169/LConn1
  _CN_192882077_330000_CN_112459307_330000/RConn1 -- T_112459307__Подстанция_330/LConn1 -- _CN_302862370_330000_CN_112459307_330000/LConn1 -- _CN_112459307_330000_CN_230015157_330000/LConn1
  _CN_192882077_330000_CN_112459307_330000/RConn2 -- T_112459307__Подстанция_330/LConn2 -- _CN_302862370_330000_CN_112459307_330000/LConn2 -- _CN_112459307_330000_CN_230015157_330000/LConn2
  _CN_192882077_330000_CN_112459307_330000/RConn3 -- T_112459307__Подстанция_330/LConn3 -- _CN_302862370_330000_CN_112459307_330000/LConn3 -- _CN_112459307_330000_CN_230015157_330000/LConn3 -- bus170/LConn1
  T_302862370__/LConn1 -- _CN_302862370_330000_CN_112459307_330000/RConn1
  T_302862370__/LConn2 -- _CN_302862370_330000_CN_112459307_330000/RConn2
  _CN_302862370_330000_CN_112459307_330000/RConn3 -- T_302862370__/LConn3 -- bus171/LConn1
  _CN_302578595_330000_CN_287216880_330000/LConn1 -- T_302578595__/LConn1 -- _CN_302578595_330000_CN_203557338_330000/LConn1
  _CN_302578595_330000_CN_287216880_330000/LConn2 -- T_302578595__/LConn2 -- _CN_302578595_330000_CN_203557338_330000/LConn2
  _CN_302578595_330000_CN_287216880_330000/LConn3 -- T_302578595__/LConn3 -- _CN_302578595_330000_CN_203557338_330000/LConn3 -- bus172/LConn1
  _CN_302578595_330000_CN_287216880_330000/RConn1 -- T_287216880_330000_Гомель_330/LConn1 -- _CN_230015157_330000_CN_287216880_330000/LConn1 -- _CN_295414241_330000_CN_287216880_330000/LConn1
  _CN_302578595_330000_CN_287216880_330000/RConn2 -- T_287216880_330000_Гомель_330/LConn2 -- _CN_230015157_330000_CN_287216880_330000/LConn2 -- _CN_295414241_330000_CN_287216880_330000/LConn2
  _CN_302578595_330000_CN_287216880_330000/RConn3 -- T_287216880_330000_Гомель_330/LConn3 -- _CN_230015157_330000_CN_287216880_330000/LConn3 -- _CN_295414241_330000_CN_287216880_330000/LConn3 -- bus173/LConn1
  "T_203557338_330000;110000;fixme_ПС_330кВ_\"Рославль\""/LConn1 -- _CN_302578595_330000_CN_203557338_330000/RConn1
  "T_203557338_330000;110000;fixme_ПС_330кВ_\"Рославль\""/LConn2 -- _CN_302578595_330000_CN_203557338_330000/RConn2
  _CN_302578595_330000_CN_203557338_330000/RConn3 -- "T_203557338_330000;110000;fixme_ПС_330кВ_\"Рославль\""/LConn3 -- bus174/LConn1
  _CN_112459307_330000_CN_230015157_330000/RConn1 -- T_230015157__/LConn1 -- _CN_230015157_330000_CN_287216880_330000/RConn1 -- _CN_230015157_330000_CN_300180022_330000/LConn1
  _CN_112459307_330000_CN_230015157_330000/RConn2 -- T_230015157__/LConn2 -- _CN_230015157_330000_CN_287216880_330000/RConn2 -- _CN_230015157_330000_CN_300180022_330000/LConn2
  _CN_112459307_330000_CN_230015157_330000/RConn3 -- T_230015157__/LConn3 -- _CN_230015157_330000_CN_287216880_330000/RConn3 -- _CN_230015157_330000_CN_300180022_330000/LConn3 -- bus175/LConn1
  _CN_243317420_330000_CN_171987005_330000/LConn1 -- T_243317420_330000_/LConn1 -- _CN_243317420_330000_CN_245414984_330000/LConn1
  _CN_243317420_330000_CN_171987005_330000/LConn2 -- T_243317420_330000_/LConn2 -- _CN_243317420_330000_CN_245414984_330000/LConn2
  _CN_243317420_330000_CN_171987005_330000/LConn3 -- T_243317420_330000_/LConn3 -- _CN_243317420_330000_CN_245414984_330000/LConn3 -- bus176/LConn1
  T_171987005_330000;110000;fixme_/LConn1 -- _CN_243317420_330000_CN_171987005_330000/RConn1
  T_171987005_330000;110000;fixme_/LConn2 -- _CN_243317420_330000_CN_171987005_330000/RConn2
  _CN_243317420_330000_CN_171987005_330000/RConn3 -- T_171987005_330000;110000;fixme_/LConn3 -- bus177/LConn1
  _CN_243317420_330000_CN_245414984_330000/RConn1 -- "T_245414984__Подстанция_330_кВ_\"Молодечно\""/LConn1 -- ВЛ_334_Молодечно___Северная_CN_245414984_330000_CN_229441506_330000/LConn1 -- _CN_283245238_330000_CN_245414984_330000/LConn1
  _CN_243317420_330000_CN_245414984_330000/RConn2 -- "T_245414984__Подстанция_330_кВ_\"Молодечно\""/LConn2 -- ВЛ_334_Молодечно___Северная_CN_245414984_330000_CN_229441506_330000/LConn2 -- _CN_283245238_330000_CN_245414984_330000/LConn2
  _CN_243317420_330000_CN_245414984_330000/RConn3 -- "T_245414984__Подстанция_330_кВ_\"Молодечно\""/LConn3 -- ВЛ_334_Молодечно___Северная_CN_245414984_330000_CN_229441506_330000/LConn3 -- bus178/LConn1 -- _CN_283245238_330000_CN_245414984_330000/LConn3
  ВЛ_330_кВ_ТЭЦ_4___Слуцк_CN_247791024_330000_CN_25465034_330000/RConn1 -- T_25465034__/LConn1 -- ВЛ_330кВ_№342_Колядичи__ТЭЦ_4_CN_25465034_330000_CN_75423694_330000/LConn1 -- ВЛ_343_ТЭЦ_4___Северная_CN_25465034_330000_CN_229441506_330000/LConn1
  ВЛ_330_кВ_ТЭЦ_4___Слуцк_CN_247791024_330000_CN_25465034_330000/RConn2 -- T_25465034__/LConn2 -- ВЛ_330кВ_№342_Колядичи__ТЭЦ_4_CN_25465034_330000_CN_75423694_330000/LConn2 -- ВЛ_343_ТЭЦ_4___Северная_CN_25465034_330000_CN_229441506_330000/LConn2
  ВЛ_330_кВ_ТЭЦ_4___Слуцк_CN_247791024_330000_CN_25465034_330000/RConn3 -- T_25465034__/LConn3 -- ВЛ_330кВ_№342_Колядичи__ТЭЦ_4_CN_25465034_330000_CN_75423694_330000/LConn3 -- ВЛ_343_ТЭЦ_4___Северная_CN_25465034_330000_CN_229441506_330000/LConn3 -- bus179/LConn1
  ВЛ_330_кВ_Гродно_Лида_CN_29428018_330000_CN_283245238_330000/LConn1 -- T_29428018_330000_ПС_330_кВ_Гродно/LConn1 -- ВЛ_330_кВ_Гродно_Гродно_Южная_CN_29428018_330000_CN_230054607_330000/LConn1 -- ВЛ_330_кВ_Гродно_Гродно_Южная_CN_29428018_330000_CN_201828730_330000/LConn1
  ВЛ_330_кВ_Гродно_Лида_CN_29428018_330000_CN_283245238_330000/LConn2 -- T_29428018_330000_ПС_330_кВ_Гродно/LConn2 -- ВЛ_330_кВ_Гродно_Гродно_Южная_CN_29428018_330000_CN_230054607_330000/LConn2 -- ВЛ_330_кВ_Гродно_Гродно_Южная_CN_29428018_330000_CN_201828730_330000/LConn2
  ВЛ_330_кВ_Гродно_Лида_CN_29428018_330000_CN_283245238_330000/LConn3 -- T_29428018_330000_ПС_330_кВ_Гродно/LConn3 -- ВЛ_330_кВ_Гродно_Гродно_Южная_CN_29428018_330000_CN_230054607_330000/LConn3 -- ВЛ_330_кВ_Гродно_Гродно_Южная_CN_29428018_330000_CN_201828730_330000/LConn3 -- bus180/LConn1
  ВЛ_330_кВ_Гродно_Лида_CN_29428018_330000_CN_283245238_330000/RConn1 -- T_283245238_330000_/LConn1 -- _CN_283245238_330000_CN_245414984_330000/RConn1
  ВЛ_330_кВ_Гродно_Лида_CN_29428018_330000_CN_283245238_330000/RConn2 -- T_283245238_330000_/LConn2 -- _CN_283245238_330000_CN_245414984_330000/RConn2
  ВЛ_330_кВ_Гродно_Лида_CN_29428018_330000_CN_283245238_330000/RConn3 -- T_283245238_330000_/LConn3 -- _CN_283245238_330000_CN_245414984_330000/RConn3 -- bus181/LConn1
  T_230054607__Барановичи_330/LConn1 -- ВЛ_330_кВ_Гродно_Гродно_Южная_CN_29428018_330000_CN_230054607_330000/RConn1
  T_230054607__Барановичи_330/LConn2 -- ВЛ_330_кВ_Гродно_Гродно_Южная_CN_29428018_330000_CN_230054607_330000/RConn2
  ВЛ_330_кВ_Гродно_Гродно_Южная_CN_29428018_330000_CN_230054607_330000/RConn3 -- T_230054607__Барановичи_330/LConn3 -- bus182/LConn1
  T_201828730_330000_/LConn1 -- ВЛ_330_кВ_Гродно_Гродно_Южная_CN_29428018_330000_CN_201828730_330000/RConn1
  T_201828730_330000_/LConn2 -- ВЛ_330_кВ_Гродно_Гродно_Южная_CN_29428018_330000_CN_201828730_330000/RConn2
  ВЛ_330_кВ_Гродно_Гродно_Южная_CN_29428018_330000_CN_201828730_330000/RConn3 -- T_201828730_330000_/LConn3 -- bus183/LConn1
  T_300180022__ГСМ_330/LConn1 -- _CN_230015157_330000_CN_300180022_330000/RConn1
  T_300180022__ГСМ_330/LConn2 -- _CN_230015157_330000_CN_300180022_330000/RConn2
  _CN_230015157_330000_CN_300180022_330000/RConn3 -- T_300180022__ГСМ_330/LConn3 -- bus184/LConn1
  ВЛ_334_Молодечно___Северная_CN_245414984_330000_CN_229441506_330000/RConn1 -- T_229441506_330000_/LConn1 -- ВЛ_426_Восточная___Северная_CN_229441506_330000_CN_405472760_330000/RConn1 -- ВЛ_343_ТЭЦ_4___Северная_CN_25465034_330000_CN_229441506_330000/RConn1
  ВЛ_334_Молодечно___Северная_CN_245414984_330000_CN_229441506_330000/RConn2 -- T_229441506_330000_/LConn2 -- ВЛ_426_Восточная___Северная_CN_229441506_330000_CN_405472760_330000/RConn2 -- ВЛ_343_ТЭЦ_4___Северная_CN_25465034_330000_CN_229441506_330000/RConn2
  ВЛ_334_Молодечно___Северная_CN_245414984_330000_CN_229441506_330000/RConn3 -- T_229441506_330000_/LConn3 -- ВЛ_426_Восточная___Северная_CN_229441506_330000_CN_405472760_330000/RConn3 -- bus185/LConn1 -- ВЛ_343_ТЭЦ_4___Северная_CN_25465034_330000_CN_229441506_330000/RConn3
  "T_75423694__ПС_\"Колядичи\""/LConn1 -- ВЛ_330кВ_№342_Колядичи__ТЭЦ_4_CN_25465034_330000_CN_75423694_330000/RConn1
  "T_75423694__ПС_\"Колядичи\""/LConn2 -- ВЛ_330кВ_№342_Колядичи__ТЭЦ_4_CN_25465034_330000_CN_75423694_330000/RConn2
  ВЛ_330кВ_№342_Колядичи__ТЭЦ_4_CN_25465034_330000_CN_75423694_330000/RConn3 -- "T_75423694__ПС_\"Колядичи\""/LConn3 -- bus186/LConn1
  T_295414241__/LConn1 -- _CN_295414241_330000_CN_287216880_330000/RConn1
  T_295414241__/LConn2 -- _CN_295414241_330000_CN_287216880_330000/RConn2
  _CN_295414241_330000_CN_287216880_330000/RConn3 -- T_295414241__/LConn3 -- bus187/LConn1
  T_293152176__/RConn1 -- L_293152176/LConn1
  T_293152176__/RConn2 -- L_293152176/LConn2
  L_293152176/LConn3 -- T_293152176__/RConn3 -- bus188/LConn1
  T_288873859__/RConn1 -- L_288873859/LConn1
  T_288873859__/RConn2 -- L_288873859/LConn2
  L_288873859/LConn3 -- T_288873859__/RConn3 -- bus189/LConn1
  T_289692683__/RConn1 -- L_289692683/LConn1
  T_289692683__/RConn2 -- L_289692683/LConn2
  L_289692683/LConn3 -- T_289692683__/RConn3 -- bus190/LConn1
  T_201916933__/RConn1 -- L_201916933/LConn1
  T_201916933__/RConn2 -- L_201916933/LConn2
  L_201916933/LConn3 -- T_201916933__/RConn3 -- bus191/LConn1
  T_89723141__ПС_110_кВ_Лозы/RConn1 -- L_89723141/LConn1
  T_89723141__ПС_110_кВ_Лозы/RConn2 -- L_89723141/LConn2
  L_89723141/LConn3 -- T_89723141__ПС_110_кВ_Лозы/RConn3 -- bus192/LConn1
  T_235777846__/RConn1 -- L_235777846/LConn1
  T_235777846__/RConn2 -- L_235777846/LConn2
  L_235777846/LConn3 -- T_235777846__/RConn3 -- bus193/LConn1
  T_222762508__/RConn1 -- L_222762508/LConn1
  T_222762508__/RConn2 -- L_222762508/LConn2
  L_222762508/LConn3 -- T_222762508__/RConn3 -- bus194/LConn1
  T_231764788_110000_ПС_Фаниполь/RConn1 -- L_231764788/LConn1
  T_231764788_110000_ПС_Фаниполь/RConn2 -- L_231764788/LConn2
  L_231764788/LConn3 -- T_231764788_110000_ПС_Фаниполь/RConn3 -- bus195/LConn1
  T_157204623_110000_/RConn1 -- L_157204623/LConn1
  T_157204623_110000_/RConn2 -- L_157204623/LConn2
  L_157204623/LConn3 -- T_157204623_110000_/RConn3 -- bus196/LConn1
  T_314244319__/RConn1 -- L_314244319/LConn1
  T_314244319__/RConn2 -- L_314244319/LConn2
  L_314244319/LConn3 -- T_314244319__/RConn3 -- bus197/LConn1
  T_314243562__/RConn1 -- L_314243562/LConn1
  T_314243562__/RConn2 -- L_314243562/LConn2
  L_314243562/LConn3 -- T_314243562__/RConn3 -- bus198/LConn1
  "T_429035693__ПС_\"Островы\""/RConn1 -- L_429035693/LConn1
  "T_429035693__ПС_\"Островы\""/RConn2 -- L_429035693/LConn2
  L_429035693/LConn3 -- "T_429035693__ПС_\"Островы\""/RConn3 -- bus199/LConn1
  "T_296016627__ПС_\"Мачулищи\""/RConn1 -- L_296016627/LConn1
  "T_296016627__ПС_\"Мачулищи\""/RConn2 -- L_296016627/LConn2
  L_296016627/LConn3 -- "T_296016627__ПС_\"Мачулищи\""/RConn3 -- bus200/LConn1
  "T_296016647__ПС_\"Кожзавод\""/RConn1 -- L_296016647/LConn1
  "T_296016647__ПС_\"Кожзавод\""/RConn2 -- L_296016647/LConn2
  L_296016647/LConn3 -- "T_296016647__ПС_\"Кожзавод\""/RConn3 -- bus201/LConn1
  T_262743896__/RConn1 -- L_262743896/LConn1
  T_262743896__/RConn2 -- L_262743896/LConn2
  L_262743896/LConn3 -- T_262743896__/RConn3 -- bus202/LConn1
  "T_59099213__ПС_\"Юго_Запад\""/RConn1 -- L_59099213/LConn1
  "T_59099213__ПС_\"Юго_Запад\""/RConn2 -- L_59099213/LConn2
  L_59099213/LConn3 -- "T_59099213__ПС_\"Юго_Запад\""/RConn3 -- bus203/LConn1
  "T_41194024__ПС_\"Курасовщина\""/RConn1 -- L_41194024/LConn1
  "T_41194024__ПС_\"Курасовщина\""/RConn2 -- L_41194024/LConn2
  L_41194024/LConn3 -- "T_41194024__ПС_\"Курасовщина\""/RConn3 -- bus204/LConn1
  "T_429148816__ПС_\"Кока_кола\""/RConn1 -- L_429148816/LConn1
  "T_429148816__ПС_\"Кока_кола\""/RConn2 -- L_429148816/LConn2
  L_429148816/LConn3 -- "T_429148816__ПС_\"Кока_кола\""/RConn3 -- bus205/LConn1
  T_310063635__/RConn1 -- L_310063635/LConn1
  T_310063635__/RConn2 -- L_310063635/LConn2
  L_310063635/LConn3 -- T_310063635__/RConn3 -- bus206/LConn1
  T_310178136__/RConn1 -- L_310178136/LConn1
  T_310178136__/RConn2 -- L_310178136/LConn2
  L_310178136/LConn3 -- T_310178136__/RConn3 -- bus207/LConn1
  T_299173918__/RConn1 -- L_299173918/LConn1
  T_299173918__/RConn2 -- L_299173918/LConn2
  L_299173918/LConn3 -- T_299173918__/RConn3 -- bus208/LConn1
  T_240568902__/RConn1 -- L_240568902/LConn1
  T_240568902__/RConn2 -- L_240568902/LConn2
  L_240568902/LConn3 -- T_240568902__/RConn3 -- bus209/LConn1
  T_287228165__/RConn1 -- L_287228165/LConn1
  T_287228165__/RConn2 -- L_287228165/LConn2
  L_287228165/LConn3 -- T_287228165__/RConn3 -- bus210/LConn1
  T_287231999__/RConn1 -- L_287231999/LConn1
  T_287231999__/RConn2 -- L_287231999/LConn2
  L_287231999/LConn3 -- T_287231999__/RConn3 -- bus211/LConn1
  T_130795400__/RConn1 -- L_130795400/LConn1
  T_130795400__/RConn2 -- L_130795400/LConn2
  L_130795400/LConn3 -- T_130795400__/RConn3 -- bus212/LConn1
  T_237040560__/RConn1 -- L_237040560/LConn1
  T_237040560__/RConn2 -- L_237040560/LConn2
  L_237040560/LConn3 -- T_237040560__/RConn3 -- bus213/LConn1
  T_302900770__/RConn1 -- L_302900770/LConn1
  T_302900770__/RConn2 -- L_302900770/LConn2
  L_302900770/LConn3 -- T_302900770__/RConn3 -- bus214/LConn1
  T_314058489__/RConn1 -- L_314058489/LConn1
  T_314058489__/RConn2 -- L_314058489/LConn2
  L_314058489/LConn3 -- T_314058489__/RConn3 -- bus215/LConn1
  T_288873564__/RConn1 -- L_288873564/LConn1
  T_288873564__/RConn2 -- L_288873564/LConn2
  L_288873564/LConn3 -- T_288873564__/RConn3 -- bus216/LConn1
  T_299211088__/RConn1 -- L_299211088/LConn1
  T_299211088__/RConn2 -- L_299211088/LConn2
  L_299211088/LConn3 -- T_299211088__/RConn3 -- bus217/LConn1
  "T_224125485__ПС_\"Волма\""/RConn1 -- L_224125485/LConn1
  "T_224125485__ПС_\"Волма\""/RConn2 -- L_224125485/LConn2
  L_224125485/LConn3 -- "T_224125485__ПС_\"Волма\""/RConn3 -- bus218/LConn1
  "T_429056529__ПС_\"Сосны\""/RConn1 -- L_429056529/LConn1
  "T_429056529__ПС_\"Сосны\""/RConn2 -- L_429056529/LConn2
  L_429056529/LConn3 -- "T_429056529__ПС_\"Сосны\""/RConn3 -- bus219/LConn1
  T_429361631__/RConn1 -- L_429361631/LConn1
  T_429361631__/RConn2 -- L_429361631/LConn2
  L_429361631/LConn3 -- T_429361631__/RConn3 -- bus220/LConn1
  T_151029302__ПС_17_«Сторожёвская»/RConn1 -- L_151029302/LConn1
  T_151029302__ПС_17_«Сторожёвская»/RConn2 -- L_151029302/LConn2
  L_151029302/LConn3 -- T_151029302__ПС_17_«Сторожёвская»/RConn3 -- bus221/LConn1
  "T_40551785__ПС_\"Уручье\""/RConn1 -- L_40551785/LConn1
  "T_40551785__ПС_\"Уручье\""/RConn2 -- L_40551785/LConn2
  L_40551785/LConn3 -- "T_40551785__ПС_\"Уручье\""/RConn3 -- bus222/LConn1
  "T_429372327__ПС_\"Дражня\""/RConn1 -- L_429372327/LConn1
  "T_429372327__ПС_\"Дражня\""/RConn2 -- L_429372327/LConn2
  L_429372327/LConn3 -- "T_429372327__ПС_\"Дражня\""/RConn3 -- bus223/LConn1
  "T_60131045__ПС_\"Озерище\""/RConn1 -- L_60131045/LConn1
  "T_60131045__ПС_\"Озерище\""/RConn2 -- L_60131045/LConn2
  L_60131045/LConn3 -- "T_60131045__ПС_\"Озерище\""/RConn3 -- bus224/LConn1
  T_300409914__/RConn1 -- L_300409914/LConn1
  T_300409914__/RConn2 -- L_300409914/LConn2
  L_300409914/LConn3 -- T_300409914__/RConn3 -- bus225/LConn1
  T_364529034__/RConn1 -- L_364529034/LConn1
  T_364529034__/RConn2 -- L_364529034/LConn2
  L_364529034/LConn3 -- T_364529034__/RConn3 -- bus226/LConn1
  T_173944054__/RConn1 -- L_173944054/LConn1
  T_173944054__/RConn2 -- L_173944054/LConn2
  L_173944054/LConn3 -- T_173944054__/RConn3 -- bus227/LConn1
  T_429929483__/RConn1 -- L_429929483/LConn1
  T_429929483__/RConn2 -- L_429929483/LConn2
  L_429929483/LConn3 -- T_429929483__/RConn3 -- bus228/LConn1
  T_301229003__/RConn1 -- L_301229003/LConn1
  T_301229003__/RConn2 -- L_301229003/LConn2
  L_301229003/LConn3 -- T_301229003__/RConn3 -- bus229/LConn1
  T_299231301__/RConn1 -- L_299231301/LConn1
  T_299231301__/RConn2 -- L_299231301/LConn2
  L_299231301/LConn3 -- T_299231301__/RConn3 -- bus230/LConn1
  T_299226289__/RConn1 -- L_299226289/LConn1
  T_299226289__/RConn2 -- L_299226289/LConn2
  L_299226289/LConn3 -- T_299226289__/RConn3 -- bus231/LConn1
  T_263648841__/RConn1 -- L_263648841/LConn1
  T_263648841__/RConn2 -- L_263648841/LConn2
  L_263648841/LConn3 -- T_263648841__/RConn3 -- bus232/LConn1
  T_268654506__/RConn1 -- L_268654506/LConn1
  T_268654506__/RConn2 -- L_268654506/LConn2
  L_268654506/LConn3 -- T_268654506__/RConn3 -- bus233/LConn1
  T_302733791__/RConn1 -- L_302733791/LConn1
  T_302733791__/RConn2 -- L_302733791/LConn2
  L_302733791/LConn3 -- T_302733791__/RConn3 -- bus234/LConn1
  T_302726346_110000_Северная/RConn1 -- L_302726346/LConn1
  T_302726346_110000_Северная/RConn2 -- L_302726346/LConn2
  L_302726346/LConn3 -- T_302726346_110000_Северная/RConn3 -- bus235/LConn1
  T_302734379__/RConn1 -- L_302734379/LConn1
  T_302734379__/RConn2 -- L_302734379/LConn2
  L_302734379/LConn3 -- T_302734379__/RConn3 -- bus236/LConn1
  T_288267865__/RConn1 -- L_288267865/LConn1
  T_288267865__/RConn2 -- L_288267865/LConn2
  L_288267865/LConn3 -- T_288267865__/RConn3 -- bus237/LConn1
  T_295775463__/RConn1 -- L_295775463/LConn1
  T_295775463__/RConn2 -- L_295775463/LConn2
  L_295775463/LConn3 -- T_295775463__/RConn3 -- bus238/LConn1
  T_289493943__РЭС/RConn1 -- L_289493943/LConn1
  T_289493943__РЭС/RConn2 -- L_289493943/LConn2
  L_289493943/LConn3 -- T_289493943__РЭС/RConn3 -- bus239/LConn1
  T_289501225__/RConn1 -- L_289501225/LConn1
  T_289501225__/RConn2 -- L_289501225/LConn2
  L_289501225/LConn3 -- T_289501225__/RConn3 -- bus240/LConn1
  "T_255157340__Stacja_elektroenergetyczna_110kV_\"Hołowczyce\""/RConn1 -- L_255157340/LConn1
  "T_255157340__Stacja_elektroenergetyczna_110kV_\"Hołowczyce\""/RConn2 -- L_255157340/LConn2
  L_255157340/LConn3 -- "T_255157340__Stacja_elektroenergetyczna_110kV_\"Hołowczyce\""/RConn3 -- bus241/LConn1
  "T_110512784__Stacja_elektroenergetyczna_110kV_\"Janów_Podlaski\""/RConn1 -- L_110512784/LConn1
  "T_110512784__Stacja_elektroenergetyczna_110kV_\"Janów_Podlaski\""/RConn2 -- L_110512784/LConn2
  L_110512784/LConn3 -- "T_110512784__Stacja_elektroenergetyczna_110kV_\"Janów_Podlaski\""/RConn3 -- bus242/LConn1
  T_310325079__ПС_110_кВ_«Копыль»/RConn1 -- L_310325079/LConn1
  T_310325079__ПС_110_кВ_«Копыль»/RConn2 -- L_310325079/LConn2
  L_310325079/LConn3 -- T_310325079__ПС_110_кВ_«Копыль»/RConn3 -- bus243/LConn1
  "T_300419261__ПС_110_кВ_\"Терасполь\""/RConn1 -- L_300419261/LConn1
  "T_300419261__ПС_110_кВ_\"Терасполь\""/RConn2 -- L_300419261/LConn2
  L_300419261/LConn3 -- "T_300419261__ПС_110_кВ_\"Терасполь\""/RConn3 -- bus244/LConn1
  T_300416246__/RConn1 -- L_300416246/LConn1
  T_300416246__/RConn2 -- L_300416246/LConn2
  L_300416246/LConn3 -- T_300416246__/RConn3 -- bus245/LConn1
  T_299972194__/RConn1 -- L_299972194/LConn1
  T_299972194__/RConn2 -- L_299972194/LConn2
  L_299972194/LConn3 -- T_299972194__/RConn3 -- bus246/LConn1
  T_299960721__/RConn1 -- L_299960721/LConn1
  T_299960721__/RConn2 -- L_299960721/LConn2
  L_299960721/LConn3 -- T_299960721__/RConn3 -- bus247/LConn1
  "T_417002086_110000_ПС_\"Корзюки\""/RConn1 -- L_417002086/LConn1
  "T_417002086_110000_ПС_\"Корзюки\""/RConn2 -- L_417002086/LConn2
  L_417002086/LConn3 -- "T_417002086_110000_ПС_\"Корзюки\""/RConn3 -- bus248/LConn1
  T_429868839__/RConn1 -- L_429868839/LConn1
  T_429868839__/RConn2 -- L_429868839/LConn2
  L_429868839/LConn3 -- T_429868839__/RConn3 -- bus249/LConn1
  T_429740435__/RConn1 -- L_429740435/LConn1
  T_429740435__/RConn2 -- L_429740435/LConn2
  L_429740435/LConn3 -- T_429740435__/RConn3 -- bus250/LConn1
  T_429148815__/RConn1 -- L_429148815/LConn1
  T_429148815__/RConn2 -- L_429148815/LConn2
  L_429148815/LConn3 -- T_429148815__/RConn3 -- bus251/LConn1
  T_301876843__/RConn1 -- L_301876843/LConn1
  T_301876843__/RConn2 -- L_301876843/LConn2
  L_301876843/LConn3 -- T_301876843__/RConn3 -- bus252/LConn1
  T_296183529__/RConn1 -- L_296183529/LConn1
  T_296183529__/RConn2 -- L_296183529/LConn2
  L_296183529/LConn3 -- T_296183529__/RConn3 -- bus253/LConn1
  "T_222038644__ПС_\"Свислочь\""/RConn1 -- L_222038644/LConn1
  "T_222038644__ПС_\"Свислочь\""/RConn2 -- L_222038644/LConn2
  L_222038644/LConn3 -- "T_222038644__ПС_\"Свислочь\""/RConn3 -- bus254/LConn1
  "T_429035699__ПС_\"СУ_ТЭЦ_5\""/RConn1 -- L_429035699/LConn1
  "T_429035699__ПС_\"СУ_ТЭЦ_5\""/RConn2 -- L_429035699/LConn2
  L_429035699/LConn3 -- "T_429035699__ПС_\"СУ_ТЭЦ_5\""/RConn3 -- bus255/LConn1
  "T_226901999__ПС_\"Руденск\""/RConn1 -- L_226901999/LConn1
  "T_226901999__ПС_\"Руденск\""/RConn2 -- L_226901999/LConn2
  L_226901999/LConn3 -- "T_226901999__ПС_\"Руденск\""/RConn3 -- bus256/LConn1
  T_299263429__/RConn1 -- L_299263429/LConn1
  T_299263429__/RConn2 -- L_299263429/LConn2
  L_299263429/LConn3 -- T_299263429__/RConn3 -- bus257/LConn1
  T_296414541__/RConn1 -- L_296414541/LConn1
  T_296414541__/RConn2 -- L_296414541/LConn2
  L_296414541/LConn3 -- T_296414541__/RConn3 -- bus258/LConn1
  T_289722224__/RConn1 -- L_289722224/LConn1
  T_289722224__/RConn2 -- L_289722224/LConn2
  L_289722224/LConn3 -- T_289722224__/RConn3 -- bus259/LConn1
  T_294809961__/RConn1 -- L_294809961/LConn1
  T_294809961__/RConn2 -- L_294809961/LConn2
  L_294809961/LConn3 -- T_294809961__/RConn3 -- bus260/LConn1
  T_287057886__/RConn1 -- L_287057886/LConn1
  T_287057886__/RConn2 -- L_287057886/LConn2
  L_287057886/LConn3 -- T_287057886__/RConn3 -- bus261/LConn1
  T_34327162__/RConn1 -- L_34327162/LConn1
  T_34327162__/RConn2 -- L_34327162/LConn2
  L_34327162/LConn3 -- T_34327162__/RConn3 -- bus262/LConn1
  T_177731028__/RConn1 -- L_177731028/LConn1
  T_177731028__/RConn2 -- L_177731028/LConn2
  L_177731028/LConn3 -- T_177731028__/RConn3 -- bus263/LConn1
  T_194912891__Stacja_elektroenergetyczna_110_15_kV_Lubień/RConn1 -- L_194912891/LConn1
  T_194912891__Stacja_elektroenergetyczna_110_15_kV_Lubień/RConn2 -- L_194912891/LConn2
  L_194912891/LConn3 -- T_194912891__Stacja_elektroenergetyczna_110_15_kV_Lubień/RConn3 -- bus264/LConn1
  T_105490801__Stacja_elektroenergetyczna_110_15_kV_Włodawa/RConn1 -- L_105490801/LConn1
  T_105490801__Stacja_elektroenergetyczna_110_15_kV_Włodawa/RConn2 -- L_105490801/LConn2
  L_105490801/LConn3 -- T_105490801__Stacja_elektroenergetyczna_110_15_kV_Włodawa/RConn3 -- bus265/LConn1
  T_230273156__/RConn1 -- L_230273156/LConn1
  T_230273156__/RConn2 -- L_230273156/LConn2
  L_230273156/LConn3 -- T_230273156__/RConn3 -- bus266/LConn1
  T_230273164_110000_Подстанция_110_кВ_Южная/RConn1 -- L_230273164/LConn1
  T_230273164_110000_Подстанция_110_кВ_Южная/RConn2 -- L_230273164/LConn2
  L_230273164/LConn3 -- T_230273164_110000_Подстанция_110_кВ_Южная/RConn3 -- bus267/LConn1
  "T_142803081__ПС_\"Заславль\""/RConn1 -- L_142803081/LConn1
  "T_142803081__ПС_\"Заславль\""/RConn2 -- L_142803081/LConn2
  L_142803081/LConn3 -- "T_142803081__ПС_\"Заславль\""/RConn3 -- bus268/LConn1
  "T_429035686__ПС_\"Мехкарьер\""/RConn1 -- L_429035686/LConn1
  "T_429035686__ПС_\"Мехкарьер\""/RConn2 -- L_429035686/LConn2
  L_429035686/LConn3 -- "T_429035686__ПС_\"Мехкарьер\""/RConn3 -- bus269/LConn1
  "T_108158175__Stacja_elektroenergetyczna_110kV_\"Wólka_Dobryńska\""/RConn1 -- L_108158175/LConn1
  "T_108158175__Stacja_elektroenergetyczna_110kV_\"Wólka_Dobryńska\""/RConn2 -- L_108158175/LConn2
  L_108158175/LConn3 -- "T_108158175__Stacja_elektroenergetyczna_110kV_\"Wólka_Dobryńska\""/RConn3 -- bus270/LConn1
  "T_248455324__ПС_\"Атлант\""/RConn1 -- L_248455324/LConn1
  "T_248455324__ПС_\"Атлант\""/RConn2 -- L_248455324/LConn2
  L_248455324/LConn3 -- "T_248455324__ПС_\"Атлант\""/RConn3 -- bus271/LConn1
  "T_248452429__ПС_\"Шабаны_2\""/RConn1 -- L_248452429/LConn1
  "T_248452429__ПС_\"Шабаны_2\""/RConn2 -- L_248452429/LConn2
  L_248452429/LConn3 -- "T_248452429__ПС_\"Шабаны_2\""/RConn3 -- bus272/LConn1
  T_227158696__/RConn1 -- L_227158696/LConn1
  T_227158696__/RConn2 -- L_227158696/LConn2
  L_227158696/LConn3 -- T_227158696__/RConn3 -- bus273/LConn1
  T_240810375__/RConn1 -- L_240810375/LConn1
  T_240810375__/RConn2 -- L_240810375/LConn2
  L_240810375/LConn3 -- T_240810375__/RConn3 -- bus274/LConn1
  T_373095383__/RConn1 -- L_373095383/LConn1
  T_373095383__/RConn2 -- L_373095383/LConn2
  L_373095383/LConn3 -- T_373095383__/RConn3 -- bus275/LConn1
  "T_300430643__ПС_110_кВ_\"Лучники\""/RConn1 -- L_300430643/LConn1
  "T_300430643__ПС_110_кВ_\"Лучники\""/RConn2 -- L_300430643/LConn2
  L_300430643/LConn3 -- "T_300430643__ПС_110_кВ_\"Лучники\""/RConn3 -- bus276/LConn1
  T_223342356__/RConn1 -- L_223342356/LConn1
  T_223342356__/RConn2 -- L_223342356/LConn2
  L_223342356/LConn3 -- T_223342356__/RConn3 -- bus277/LConn1
  T_409058996__/RConn1 -- L_409058996/LConn1
  T_409058996__/RConn2 -- L_409058996/LConn2
  L_409058996/LConn3 -- T_409058996__/RConn3 -- bus278/LConn1
  T_232431375__/RConn1 -- L_232431375/LConn1
  T_232431375__/RConn2 -- L_232431375/LConn2
  L_232431375/LConn3 -- T_232431375__/RConn3 -- bus279/LConn1
  T_235391296__/RConn1 -- L_235391296/LConn1
  T_235391296__/RConn2 -- L_235391296/LConn2
  L_235391296/LConn3 -- T_235391296__/RConn3 -- bus280/LConn1
  "T_275034427__ПС_\"Красная_Слобода\""/RConn1 -- L_275034427/LConn1
  "T_275034427__ПС_\"Красная_Слобода\""/RConn2 -- L_275034427/LConn2
  L_275034427/LConn3 -- "T_275034427__ПС_\"Красная_Слобода\""/RConn3 -- bus281/LConn1
  T_309889740__/RConn1 -- L_309889740/LConn1
  T_309889740__/RConn2 -- L_309889740/LConn2
  L_309889740/LConn3 -- T_309889740__/RConn3 -- bus282/LConn1
  T_271931809__/RConn1 -- L_271931809/LConn1
  T_271931809__/RConn2 -- L_271931809/LConn2
  L_271931809/LConn3 -- T_271931809__/RConn3 -- bus283/LConn1
  T_296408783__/RConn1 -- L_296408783/LConn1
  T_296408783__/RConn2 -- L_296408783/LConn2
  L_296408783/LConn3 -- T_296408783__/RConn3 -- bus284/LConn1
  T_230054609__/RConn1 -- L_230054609/LConn1
  T_230054609__/RConn2 -- L_230054609/LConn2
  L_230054609/LConn3 -- T_230054609__/RConn3 -- bus285/LConn1
  T_298978939__/RConn1 -- L_298978939/LConn1
  T_298978939__/RConn2 -- L_298978939/LConn2
  L_298978939/LConn3 -- T_298978939__/RConn3 -- bus286/LConn1
  T_280269221__/RConn1 -- L_280269221/LConn1
  T_280269221__/RConn2 -- L_280269221/LConn2
  L_280269221/LConn3 -- T_280269221__/RConn3 -- bus287/LConn1
  T_173944047__/RConn1 -- L_173944047/LConn1
  T_173944047__/RConn2 -- L_173944047/LConn2
  L_173944047/LConn3 -- T_173944047__/RConn3 -- bus288/LConn1
  T_311242021__/RConn1 -- L_311242021/LConn1
  T_311242021__/RConn2 -- L_311242021/LConn2
  L_311242021/LConn3 -- T_311242021__/RConn3 -- bus289/LConn1
  T_192951026__/RConn1 -- L_192951026/LConn1
  T_192951026__/RConn2 -- L_192951026/LConn2
  L_192951026/LConn3 -- T_192951026__/RConn3 -- bus290/LConn1
  T_168120565__/RConn1 -- L_168120565/LConn1
  T_168120565__/RConn2 -- L_168120565/LConn2
  L_168120565/LConn3 -- T_168120565__/RConn3 -- bus291/LConn1
  T_199487387__/RConn1 -- L_199487387/LConn1
  T_199487387__/RConn2 -- L_199487387/LConn2
  L_199487387/LConn3 -- T_199487387__/RConn3 -- bus292/LConn1
  T_223761142__ПС_110_кВ_Гродненская_ГЭС/RConn1 -- L_223761142/LConn1
  T_223761142__ПС_110_кВ_Гродненская_ГЭС/RConn2 -- L_223761142/LConn2
  L_223761142/LConn3 -- T_223761142__ПС_110_кВ_Гродненская_ГЭС/RConn3 -- bus293/LConn1
  T_177731027__/RConn1 -- L_177731027/LConn1
  T_177731027__/RConn2 -- L_177731027/LConn2
  L_177731027/LConn3 -- T_177731027__/RConn3 -- bus294/LConn1
  "T_52763915__ПС_\"Лошица\""/RConn1 -- L_52763915/LConn1
  "T_52763915__ПС_\"Лошица\""/RConn2 -- L_52763915/LConn2
  L_52763915/LConn3 -- "T_52763915__ПС_\"Лошица\""/RConn3 -- bus295/LConn1
  T_143993676__ПС_Минский_камвольный_комбинат/RConn1 -- L_143993676/LConn1
  T_143993676__ПС_Минский_камвольный_комбинат/RConn2 -- L_143993676/LConn2
  L_143993676/LConn3 -- T_143993676__ПС_Минский_камвольный_комбинат/RConn3 -- bus296/LConn1
  T_325933845__/RConn1 -- L_325933845/LConn1
  T_325933845__/RConn2 -- L_325933845/LConn2
  L_325933845/LConn3 -- T_325933845__/RConn3 -- bus297/LConn1
  T_166169945__/RConn1 -- L_166169945/LConn1
  T_166169945__/RConn2 -- L_166169945/LConn2
  L_166169945/LConn3 -- T_166169945__/RConn3 -- bus298/LConn1
  T_230059305_110000_Осташковичи/RConn1 -- L_230059305/LConn1
  T_230059305_110000_Осташковичи/RConn2 -- L_230059305/LConn2
  L_230059305/LConn3 -- T_230059305_110000_Осташковичи/RConn3 -- bus299/LConn1
  T_366740253__/RConn1 -- L_366740253/LConn1
  T_366740253__/RConn2 -- L_366740253/LConn2
  L_366740253/LConn3 -- T_366740253__/RConn3 -- bus300/LConn1
  T_262762815__/RConn1 -- L_262762815/LConn1
  T_262762815__/RConn2 -- L_262762815/LConn2
  L_262762815/LConn3 -- T_262762815__/RConn3 -- bus301/LConn1
  T_282201051__Якимова_Слобода/RConn1 -- L_282201051/LConn1
  T_282201051__Якимова_Слобода/RConn2 -- L_282201051/LConn2
  L_282201051/LConn3 -- T_282201051__Якимова_Слобода/RConn3 -- bus302/LConn1
  T_282200754_110000_Забродье/RConn1 -- L_282200754/LConn1
  T_282200754_110000_Забродье/RConn2 -- L_282200754/LConn2
  L_282200754/LConn3 -- T_282200754_110000_Забродье/RConn3 -- bus303/LConn1
  T_286434280__/RConn1 -- L_286434280/LConn1
  T_286434280__/RConn2 -- L_286434280/LConn2
  L_286434280/LConn3 -- T_286434280__/RConn3 -- bus304/LConn1
  T_300183354__/RConn1 -- L_300183354/LConn1
  T_300183354__/RConn2 -- L_300183354/LConn2
  L_300183354/LConn3 -- T_300183354__/RConn3 -- bus305/LConn1
  T_300236667__/RConn1 -- L_300236667/LConn1
  T_300236667__/RConn2 -- L_300236667/LConn2
  L_300236667/LConn3 -- T_300236667__/RConn3 -- bus306/LConn1
  T_108689220__/RConn1 -- L_108689220/LConn1
  T_108689220__/RConn2 -- L_108689220/LConn2
  L_108689220/LConn3 -- T_108689220__/RConn3 -- bus307/LConn1
  T_295351112_330000_/RConn1 -- L_295351112/LConn1
  T_295351112_330000_/RConn2 -- L_295351112/LConn2
  L_295351112/LConn3 -- T_295351112_330000_/RConn3 -- bus308/LConn1
  T_168037760__/RConn1 -- L_168037760/LConn1
  T_168037760__/RConn2 -- L_168037760/LConn2
  L_168037760/LConn3 -- T_168037760__/RConn3 -- bus309/LConn1
  T_293851177__/RConn1 -- L_293851177/LConn1
  T_293851177__/RConn2 -- L_293851177/LConn2
  L_293851177/LConn3 -- T_293851177__/RConn3 -- bus310/LConn1
  T_276283812__/RConn1 -- L_276283812/LConn1
  T_276283812__/RConn2 -- L_276283812/LConn2
  L_276283812/LConn3 -- T_276283812__/RConn3 -- bus311/LConn1
  T_293845492__/RConn1 -- L_293845492/LConn1
  T_293845492__/RConn2 -- L_293845492/LConn2
  L_293845492/LConn3 -- T_293845492__/RConn3 -- bus312/LConn1
  T_88831410__/RConn1 -- L_88831410/LConn1
  T_88831410__/RConn2 -- L_88831410/LConn2
  L_88831410/LConn3 -- T_88831410__/RConn3 -- bus313/LConn1
  T_194911376__Stacja_elektroenergetyczna_110_15_kV_Macoszyn/RConn1 -- L_194911376/LConn1
  T_194911376__Stacja_elektroenergetyczna_110_15_kV_Macoszyn/RConn2 -- L_194911376/LConn2
  L_194911376/LConn3 -- T_194911376__Stacja_elektroenergetyczna_110_15_kV_Macoszyn/RConn3 -- bus314/LConn1
  "T_25686883__ПС_\"Сухарево\""/RConn1 -- L_25686883/LConn1
  "T_25686883__ПС_\"Сухарево\""/RConn2 -- L_25686883/LConn2
  L_25686883/LConn3 -- "T_25686883__ПС_\"Сухарево\""/RConn3 -- bus315/LConn1
  "T_264555597__ПС_\"Ждановичи\""/RConn1 -- L_264555597/LConn1
  "T_264555597__ПС_\"Ждановичи\""/RConn2 -- L_264555597/LConn2
  L_264555597/LConn3 -- "T_264555597__ПС_\"Ждановичи\""/RConn3 -- bus316/LConn1
  T_394798987__/RConn1 -- L_394798987/LConn1
  T_394798987__/RConn2 -- L_394798987/LConn2
  L_394798987/LConn3 -- T_394798987__/RConn3 -- bus317/LConn1
  "T_399298484_110000_ПС_\"Завод_запасных_частей\""/RConn1 -- L_399298484/LConn1
  "T_399298484_110000_ПС_\"Завод_запасных_частей\""/RConn2 -- L_399298484/LConn2
  L_399298484/LConn3 -- "T_399298484_110000_ПС_\"Завод_запасных_частей\""/RConn3 -- bus318/LConn1
  T_39890905__/RConn1 -- L_39890905/LConn1
  T_39890905__/RConn2 -- L_39890905/LConn2
  L_39890905/LConn3 -- T_39890905__/RConn3 -- bus319/LConn1
  T_29128697__ПС_110_кВ_Занеманская/RConn1 -- L_29128697/LConn1
  T_29128697__ПС_110_кВ_Занеманская/RConn2 -- L_29128697/LConn2
  L_29128697/LConn3 -- T_29128697__ПС_110_кВ_Занеманская/RConn3 -- bus320/LConn1
  "T_229441505__ПС_\"Вишневка\""/RConn1 -- L_229441505/LConn1
  "T_229441505__ПС_\"Вишневка\""/RConn2 -- L_229441505/LConn2
  L_229441505/LConn3 -- "T_229441505__ПС_\"Вишневка\""/RConn3 -- bus321/LConn1
  T_300347040_330000_/RConn1 -- L_300347040/LConn1
  T_300347040_330000_/RConn2 -- L_300347040/LConn2
  L_300347040/LConn3 -- T_300347040_330000_/RConn3 -- bus322/LConn1
  T_230059284__/RConn1 -- L_230059284/LConn1
  T_230059284__/RConn2 -- L_230059284/LConn2
  L_230059284/LConn3 -- T_230059284__/RConn3 -- bus323/LConn1
  T_264617753__РЭС/RConn1 -- L_264617753/LConn1
  T_264617753__РЭС/RConn2 -- L_264617753/LConn2
  L_264617753/LConn3 -- T_264617753__РЭС/RConn3 -- bus324/LConn1
  "T_216254873_220000;110000_Stacja_elektroenergetyczna_\"Białystok\"_220_110_kV"/RConn1 -- L_216254873/LConn1
  "T_216254873_220000;110000_Stacja_elektroenergetyczna_\"Białystok\"_220_110_kV"/RConn2 -- L_216254873/LConn2
  L_216254873/LConn3 -- "T_216254873_220000;110000_Stacja_elektroenergetyczna_\"Białystok\"_220_110_kV"/RConn3 -- bus325/LConn1
  T_129510527__/RConn1 -- L_129510527/LConn1
  T_129510527__/RConn2 -- L_129510527/LConn2
  L_129510527/LConn3 -- T_129510527__/RConn3 -- bus326/LConn1
  T_148660895__P_C_220_kV_BREST_2/RConn1 -- L_148660895/LConn1
  T_148660895__P_C_220_kV_BREST_2/RConn2 -- L_148660895/LConn2
  L_148660895/LConn3 -- T_148660895__P_C_220_kV_BREST_2/RConn3 -- bus327/LConn1
  T_296423596__/RConn1 -- L_296423596/LConn1
  T_296423596__/RConn2 -- L_296423596/LConn2
  L_296423596/LConn3 -- T_296423596__/RConn3 -- bus328/LConn1
  T_299839754__/RConn1 -- L_299839754/LConn1
  T_299839754__/RConn2 -- L_299839754/LConn2
  L_299839754/LConn3 -- T_299839754__/RConn3 -- bus329/LConn1
  "T_232797676__ПС_330_\"Калийная\""/RConn1 -- L_232797676/LConn1
  "T_232797676__ПС_330_\"Калийная\""/RConn2 -- L_232797676/LConn2
  L_232797676/LConn3 -- "T_232797676__ПС_330_\"Калийная\""/RConn3 -- bus330/LConn1
  "T_429151634__ПС_\"Борисов\""/RConn1 -- L_429151634/LConn1
  "T_429151634__ПС_\"Борисов\""/RConn2 -- L_429151634/LConn2
  L_429151634/LConn3 -- "T_429151634__ПС_\"Борисов\""/RConn3 -- bus331/LConn1
  "T_405472760__ПС_330_110_10_кВ_\"Восточная\""/RConn1 -- L_405472760/LConn1
  "T_405472760__ПС_330_110_10_кВ_\"Восточная\""/RConn2 -- L_405472760/LConn2
  L_405472760/LConn3 -- "T_405472760__ПС_330_110_10_кВ_\"Восточная\""/RConn3 -- bus332/LConn1
  T_112459307__Подстанция_330/RConn1 -- L_112459307/LConn1
  T_112459307__Подстанция_330/RConn2 -- L_112459307/LConn2
  L_112459307/LConn3 -- T_112459307__Подстанция_330/RConn3 -- bus333/LConn1
  T_302862370__/RConn1 -- L_302862370/LConn1
  T_302862370__/RConn2 -- L_302862370/LConn2
  L_302862370/LConn3 -- T_302862370__/RConn3 -- bus334/LConn1
  T_302578595__/RConn1 -- L_302578595/LConn1
  T_302578595__/RConn2 -- L_302578595/LConn2
  L_302578595/LConn3 -- T_302578595__/RConn3 -- bus335/LConn1
  "T_203557338_330000;110000;fixme_ПС_330кВ_\"Рославль\""/RConn1 -- L_203557338/LConn1
  "T_203557338_330000;110000;fixme_ПС_330кВ_\"Рославль\""/RConn2 -- L_203557338/LConn2
  L_203557338/LConn3 -- "T_203557338_330000;110000;fixme_ПС_330кВ_\"Рославль\""/RConn3 -- bus336/LConn1
  T_230015157__/RConn1 -- L_230015157/LConn1
  T_230015157__/RConn2 -- L_230015157/LConn2
  L_230015157/LConn3 -- T_230015157__/RConn3 -- bus337/LConn1
  T_243317420_330000_/RConn1 -- L_243317420/LConn1
  T_243317420_330000_/RConn2 -- L_243317420/LConn2
  L_243317420/LConn3 -- T_243317420_330000_/RConn3 -- bus338/LConn1
  T_25465034__/RConn1 -- L_25465034/LConn1
  T_25465034__/RConn2 -- L_25465034/LConn2
  L_25465034/LConn3 -- T_25465034__/RConn3 -- bus339/LConn1
  T_29428018_330000_ПС_330_кВ_Гродно/RConn1 -- L_29428018/LConn1
  T_29428018_330000_ПС_330_кВ_Гродно/RConn2 -- L_29428018/LConn2
  L_29428018/LConn3 -- T_29428018_330000_ПС_330_кВ_Гродно/RConn3 -- bus340/LConn1
  T_300180022__ГСМ_330/RConn1 -- L_300180022/LConn1
  T_300180022__ГСМ_330/RConn2 -- L_300180022/LConn2
  L_300180022/LConn3 -- T_300180022__ГСМ_330/RConn3 -- bus341/LConn1
  "T_75423694__ПС_\"Колядичи\""/RConn1 -- L_75423694/LConn1
  "T_75423694__ПС_\"Колядичи\""/RConn2 -- L_75423694/LConn2
  L_75423694/LConn3 -- "T_75423694__ПС_\"Колядичи\""/RConn3 -- bus342/LConn1
  T_295414241__/RConn1 -- L_295414241/LConn1
  T_295414241__/RConn2 -- L_295414241/LConn2
  L_295414241/LConn3 -- T_295414241__/RConn3 -- bus343/LConn1
